simulink library "outp"  (R2021b)
settings: Solver=VariableStepAuto  StartTime=0.0  StopTime=10.0  RelTol=1e-3
undefined symbols (not defined in the file): ENUM_PMMMODE_CHARGE, ENUM_PMMMODE_IDLE, ENUM_PMMMODE_INITIALIZE, ENUM_PMMMODE_POWERDOWN, ENUM_PMMMODE_SLEEP, Left, outp, slcm, TRUE
libraries: FVT_lib x1177, hcu_lib x4, simulink x1
(part 5 of 11)

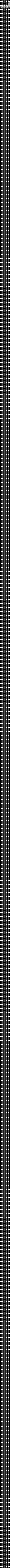
== system outp/OUTP/outpmodule ==
  VACC_HVTHCMSysAvail_enum : Inport
  VACC_LVBattVoltSta_enum : Inport  Port=2
  VACC_VehHVPwrAvail4THCM_W : Inport  Port=3
  VAPM_VehSpeed_kph : Inport  Port=4
  VAPM_VehSpeedTimeOut_flg : Inport  Port=5
  VAPM_FSOffSw_enum : Inport  Port=6
  VAPM_FSOffSwTimeOut_flg : Inport  Port=7
  VAPM_ChrgPlugSta_enum : Inport  Port=8
  VAPM_PASDRMR_cm : Inport  Port=9
  VAPM_PASDRML_cm : Inport  Port=10
  VAPM_PASDRCR_cm : Inport  Port=11
  VAPM_PASDRCL_cm : Inport  Port=12
  VAPM_PASDFMR_cm : Inport  Port=13
  VAPM_PASDFML_cm : Inport  Port=14
  VAPM_PASDFCR_cm : Inport  Port=15
  VAPM_PASDFCL_cm : Inport  Port=16
  VAPM_APSDRLR_cm : Inport  Port=17
  VAPM_APSDRLL_cm : Inport  Port=18
  VAPM_APSDFLR_cm : Inport  Port=19
  VAPM_APSDFLL_cm : Inport  Port=20
  VAPM_PASAFCL_enum : Inport  Port=21
  VAPM_PASARMR_enum : Inport  Port=22
  VAPM_PASARML_enum : Inport  Port=23
  VAPM_PASARCR_enum : Inport  Port=24
  VAPM_PASARCL_enum : Inport  Port=25
  VAPM_PASAFMR_enum : Inport  Port=26
  VAPM_PASAFML_enum : Inport  Port=27
  VAPM_PASAFCR_enum : Inport  Port=28
  VAPM_USSStaRMR_flg : Inport  Port=29
  VAPM_USSStaRML_flg : Inport  Port=30
  VAPM_USSStaRLR_flg : Inport  Port=31
  VAPM_USSStaRLL_flg : Inport  Port=32
  VAPM_USSStaRCR_flg : Inport  Port=33
  VAPM_USSStaRCL_flg : Inport  Port=34
  VAPM_USSStaFMR_flg : Inport  Port=35
  VAPM_USSStaFML_flg : Inport  Port=36
  VAPM_USSStaFLR_flg : Inport  Port=37
  VAPM_USSStaFLL_flg : Inport  Port=38
  VAPM_USSStaFCR_flg : Inport  Port=39
  VAPM_USSStaFCL_flg : Inport  Port=40
  VAPM_Chime_enum : Inport  Port=41
  VAPM_SNSRLayout_enum : Inport  Port=42
  VAPM_StaFSya_flg : Inport  Port=43
  VAPM_ModOperation_enum : Inport  Port=44
  VAPM_BrkPedalPos_pct : Inport  Port=45
  VAPM_BrkPedalPosTimeOut_flg : Inport  Port=46
  VAPM_LFRawWhlSpeed_kph : Inport  Port=47
  VAPM_LFRawWhlSpeedTimeOut_flg : Inport  Port=48
  VAPM_RFRawWhlSpeed_kph : Inport  Port=49
  VAPM_RFRawWhlSpeedTimeOut_flg : Inport  Port=50
  VAPM_LRRawWhlSpeed_kph : Inport  Port=51
  VAPM_LRRawWhlSpeedTimeOut_flg : Inport  Port=52
  VAPM_RRRawWhlSpeed_kph : Inport  Port=53
  VAPM_RRRawWhlSpeedTimeOut_flg : Inport  Port=54
  VAPM_LFRawWhlSpeedV_flg : Inport  Port=55
  VAPM_LFRawWhlSpeedVTimeOut_flg : Inport  Port=56
  VAPM_RFRawWhlSpeedV_flg : Inport  Port=57
  VAPM_RFRawWhlSpeedVTimeOut_flg : Inport  Port=58
  VAPM_LRRawWhlSpeedV_flg : Inport  Port=59
  VAPM_LRRawWhlSpeedVTimeOut_flg : Inport  Port=60
  VAPM_RRRawWhlSpeedV_flg : Inport  Port=61
  VAPM_RRRawWhlSpeedVTimeOut_flg : Inport  Port=62
  VAPM_LFWhlRotDir_enum : Inport  Port=63
  VAPM_LFWhlRotDirTimeOut_flg : Inport  Port=64
  VAPM_RFWhlRotDir_enum : Inport  Port=65
  VAPM_RFWhlRotDirTimeOut_flg : Inport  Port=66
  VAPM_LRWhlRotDir_enum : Inport  Port=67
  VAPM_LRWhlRotDirTimeOut_flg : Inport  Port=68
  VAPM_RRWhlRotDir_enum : Inport  Port=69
  VAPM_RRWhlRotDirTimeOut_flg : Inport  Port=70
  VAPM_LFPulseCountV_flg : Inport  Port=71
  VAPM_LFPulseCountVTimeOut_flg : Inport  Port=72
  VAPM_RFPulseCountV_flg : Inport  Port=73
  VAPM_RFPulseCountVTimeOut_flg : Inport  Port=74
  VAPM_LRPulseCountV_flg : Inport  Port=75
  VAPM_LRPulseCountVTimeOut_flg : Inport  Port=76
  VAPM_RRPulseCountV_flg : Inport  Port=77
  VAPM_RRPulseCountVTimeOut_flg : Inport  Port=78
  VAPM_LFPulseCount_enum : Inport  Port=79
  VAPM_LFPulseCountTimeOut_flg : Inport  Port=80
  VAPM_RFPulseCount_enum : Inport  Port=81
  VAPM_RFPulseCountTimeOut_flg : Inport  Port=82
  VAPM_LRPulseCount_enum : Inport  Port=83
  VAPM_LRPulseCountTimeOut_flg : Inport  Port=84
  VAPM_RRPulseCount_enum : Inport  Port=85
  VAPM_RRPulseCountTimeOut_flg : Inport  Port=86
  VAPM_ShifterHandleCmd_enum : Inport  Port=87
  VAPM_ShifterHandleCmdTimeOut_flg : Inport  Port=88
  VAPM_DriIntend_enum : Inport  Port=89
  VAPM_DriIntendTimeOut_flg : Inport  Port=90
  VAPM_EPSAOIControl_enum : Inport  Port=91
  VAPM_EPSAOIControlTimeOut_flg : Inport  Port=92
  VAPM_SASAngle_Deg : Inport  Port=93
  VAPM_SASAngleTimeOut_flg : Inport  Port=94
  VAPM_SASSpeed_degps : Inport  Port=95
  VAPM_SASSpeedTimeOut_flg : Inport  Port=96
  VAPM_SASSpeedValid_flg : Inport  Port=97
  VAPM_SASSpeedValidTimeOut_flg : Inport  Port=98
  VAPM_SASCAL_flg : Inport  Port=99
  VAPM_SASCALTimeOut_flg : Inport  Port=100
  VAPM_SASV_flg : Inport  Port=101
  VAPM_SASVTimeOut_flg : Inport  Port=102
  VAPM_GRADE_Deg : Inport  Port=103
  VAPM_GRADETimeOut_flg : Inport  Port=104
  VAPM_YawRate_degps : Inport  Port=105
  VAPM_YawRateTimeOut_flg : Inport  Port=106
  VAPM_LatAccel_Gps : Inport  Port=107
  VAPM_LatAccelTimeOut_flg : Inport  Port=108
  VAPM_LongAccel_Gps : Inport  Port=109
  VAPM_LongAccelTimeOut_flg : Inport  Port=110
  VAPM_MCPressure_bar : Inport  Port=111
  VAPM_MCPressureTimeOut_flg : Inport  Port=112
  VAPM_YawRateV_flg : Inport  Port=113
  VAPM_YawRateVTimeOut_flg : Inport  Port=114
  VAPM_LatAccelV_flg : Inport  Port=115
  VAPM_LatAccelVTimeOut_flg : Inport  Port=116
  VAPM_LongAccelV_flg : Inport  Port=117
  VAPM_LongAccelVTimeOut_flg : Inport  Port=118
  VAPM_MCPressureV_bar : Inport  Port=119
  VAPM_MCPressureVTimeOut_flg : Inport  Port=120
  VAPM_BrkSwSta_flg : Inport  Port=121
  VAPM_BrkSwStaTimeOut_flg : Inport  Port=122
  VAPM_BrkSwV_flg : Inport  Port=123
  VAPM_BrkSwVTimeOut_flg : Inport  Port=124
  VAPM_ESCStandstill_flg : Inport  Port=125
  VAPM_ESCStandstillTimeOut_flg : Inport  Port=126
  VAPM_ESCAPSSta_enum : Inport  Port=127
  VAPM_ESCAPSStaTimeOut_flg : Inport  Port=128
  VAPM_EPBExtReleaseAvail_flg : Inport  Port=129
  VAPM_EPBExtReleaseAvailTimeOut_flg : Inport  Port=130
  VAPM_EPBExtApplyAvail_flg : Inport  Port=131
  VAPM_EPBExtApplyAvailTimeOut_flg : Inport  Port=132
  VAPM_EPBErrSta_enum : Inport  Port=133
  VAPM_EPBErrStaTimeOut_flg : Inport  Port=134
  VAPM_EPBSta_enum : Inport  Port=135
  VAPM_EPBStaTimeOut_flg : Inport  Port=136
  VAPM_AVMparkingcancel_enum : Inport  Port=137
  VAPM_AVMparkingcancelTimeOut_flg : Inport  Port=138
  VAPM_AVMparkingexcute_enum : Inport  Port=139
  VAPM_AVMparkingexcuteTimeOut_flg : Inport  Port=140
  VAPM_AVMParkingmode_enum : Inport  Port=141
  VAPM_AVMParkingmodeTimeOut_flg : Inport  Port=142
  VAPM_AVMErrSTA_flg : Inport  Port=143
  VAPM_AVMErrSTATimeOut_flg : Inport  Port=144
  VAPM_IVIStatus_flg : Inport  Port=145
  VAPM_IVIStatusTimeOut_flg : Inport  Port=146
  VAPM_CAASSw_enum : Inport  Port=147
  VAPM_CAASSwTimeOut_flg : Inport  Port=148
  VAPM_IVIScreen_enum : Inport  Port=149
  VAPM_IVIScreenTimeOut_flg : Inport  Port=150
  VAPM_ABSActive_flg : Inport  Port=151
  VAPM_ABSActiveTimeOut_flg : Inport  Port=152
  VAPM_TCSActive_flg : Inport  Port=153
  VAPM_TCSActiveTimeOut_flg : Inport  Port=154
  VAPM_DriverSeatBeltCmd_flg : Inport  Port=155
  VAPM_DriverSeatBeltCmdTimeOut_flg : Inport  Port=156
  VAPM_APSProgressPCT_pct : Inport  Port=157
  VAPM_APSRQDisplay_enum : Inport  Port=158
  VAPM_APSSWVer_enum : Inport  Port=159
  VAPM_APSHWVer_enum : Inport  Port=160
  VAPM_APSExitCondition_enum : Inport  Port=161
  VAPM_APSAngleTarget_Deg : Inport  Port=162
  VAPM_APSVRqEPASCtrl_flg : Inport  Port=163
  VAPM_APSRqEPASCtrl_flg : Inport  Port=164
  VAPM_CAASSta_enum : Inport  Port=165
  VAPM_DKCPDkeyAreaRAPSSta_enum : Inport  Port=166
  VAPM_DKCParkingModeCmd_enum : Inport  Port=167
  VAPM_PUIDLowPower_flg : Inport  Port=168
  VAPM_CAASVMCReqA_flg : Inport  Port=169
  VAPM_APSShiftPosnReq_enum : Inport  Port=170
  VAPM_APSSpeedCMD_kph : Inport  Port=171
  VAPM_APSVMCReqA_flg : Inport  Port=172
  VAPM_RAPSBCMLamp_enum : Inport  Port=173
  VAPM_RAPSBCMLockReq_flg : Inport  Port=174
  VAPM_APSPwrReq_enum : Inport  Port=175
  VAPM_RAPSErrWarnSta_enum : Inport  Port=176
  VAPM_RAPSErrLv1_flg : Inport  Port=177
  VAPM_IVIUserTakeOverAPSSta_flg : Inport  Port=178
  VBCM_AntitheftSta_enum : Inport  Port=179
  VBCM_TailgateRemote_enum : Inport  Port=180
  VBCM_HornCtrl_flg : Inport  Port=181
  VBCM_AllDoorSW_flg : Inport  Port=182
  VBCM_BCMDoorLockSta_flg : Inport  Port=183
  VBCM_AntitheftSeatFlod_flg : Inport  Port=184
  VBCM_HoodSW_flg : Inport  Port=185
  VBCM_TailgateSW_flg : Inport  Port=186
  VBCM_DrDoorSW_flg : Inport  Port=187
  VBCM_PsDoorSW_flg : Inport  Port=188
  VBCM_RLDoorSW_flg : Inport  Port=189
  VBCM_RRDoorSW_flg : Inport  Port=190
  VBCM_LockSetting_flg : Inport  Port=191
  VBCM_FrChargingDoorCtrl_enum : Inport  Port=192
  VBCM_RrChargingDoorCtrl_enum : Inport  Port=193
  VBCM_CrashDetd_flg : Inport  Port=194
  VBCM_CTDCtrl_enum : Inport  Port=195
  VBCM_DoorLockIND_flg : Inport  Port=196
  VBCM_CTDLockSW_flg : Inport  Port=197
  VBCM_Dimmer_pct : Inport  Port=198
  VBCM_DimmerEN_flg : Inport  Port=199
  VBCM_PosLamp_flg : Inport  Port=200
  VBCM_LBeam_flg : Inport  Port=201
  VBCM_HBeam_flg : Inport  Port=202
  VBCM_RrFogLamp_flg : Inport  Port=203
  VBCM_BrakeLamp_flg : Inport  Port=204
  VBCM_ReverseLamp_flg : Inport  Port=205
  VBCM_LDRL_flg : Inport  Port=206
  VBCM_RDRL_flg : Inport  Port=207
  VBCM_LBSD_flg : Inport  Port=208
  VBCM_RBSD_flg : Inport  Port=209
  VBCM_HazardSW_flg : Inport  Port=210
  VBCM_LTurnLP_flg : Inport  Port=211
  VBCM_RTurnLP_flg : Inport  Port=212
  VBCM_BCMBuzzerReq_flg : Inport  Port=213
  VBCM_MirrorCtrl_enum : Inport  Port=214
  VBCM_MirrorDefog_flg : Inport  Port=215
  VBCM_RrDefog_flg : Inport  Port=216
  VBCM_RoomLampH_flg : Inport  Port=217
  VBCM_RoomLampL_flg : Inport  Port=218
  VBCM_TrunkRel_flg : Inport  Port=219
  VBCM_TailgateHDSW_flg : Inport  Port=220
  VBCM_FrWiperL_flg : Inport  Port=221
  VBCM_FrWiperH_flg : Inport  Port=222
  VBCM_RrWiper_flg : Inport  Port=223
  VBCM_WasherCtrl_enum : Inport  Port=224
  VBCM_WiperFixMode_flg : Inport  Port=225
  VBCM_AmbLightBreath1_enum : Inport  Port=226
  VBCM_AmbLightBreath2_enum : Inport  Port=227
  VBCM_AmbLightBreath3_enum : Inport  Port=228
  VBCM_AmbLightBreath4_enum : Inport  Port=229
  VBCM_AmbLightBreath5_enum : Inport  Port=230
  VBCM_AmbLightBreath6_enum : Inport  Port=231
  VBCM_AmbLightBrightness1_enum : Inport  Port=232
  VBCM_AmbLightBrightness2_enum : Inport  Port=233
  VBCM_AmbLightBrightness3_enum : Inport  Port=234
  VBCM_AmbLightBrightness4_enum : Inport  Port=235
  VBCM_AmbLightBrightness5_enum : Inport  Port=236
  VBCM_AmbLightBrightness6_enum : Inport  Port=237
  VBCM_AmbLightColor1_enum : Inport  Port=238
  VBCM_AmbLightColor2_enum : Inport  Port=239
  VBCM_AmbLightColor3_enum : Inport  Port=240
  VBCM_AmbLightColor4_enum : Inport  Port=241
  VBCM_AmbLightColor5_enum : Inport  Port=242
  VBCM_AmbLightColor6_enum : Inport  Port=243
  VBCM_LampPwr_flg : Inport  Port=244
  VBCM_SPTGDet_flg : Inport  Port=245
  VBCM_APSOpenPTG_flg : Inport  Port=246
  VBCM_FollowMe_flg : Inport  Port=247
  VBCM_IVIRST_flg : Inport  Port=248
  VBCM_CountAlarm_enum : Inport  Port=249
  VBCM_MFSWTri_flg : Inport  Port=250
  VBCM_MirrorFlodPos_flg : Inport  Port=251
  VBCM_FuelDoorPos_flg : Inport  Port=252
  VBCM_MFRDNBrightReq_pct : Inport  Port=253
  VBCM_PTGInnerSW2_enum : Inport  Port=254
  VBCM_DrvWdwCtrlCmd_pct : Inport  Port=255
  VBCM_PasWdwCtrlCmd_pct : Inport  Port=256
  VBCM_DrRWdwCtrlCmd_pct : Inport  Port=257
  VBCM_PsRWdwCtrlCmd_pct : Inport  Port=258
  VBCM_APMDoorControlSta_flg : Inport  Port=259
  VBCM_AmbFunEN_flg : Inport  Port=260
  VBCM_AmbWelEN_flg : Inport  Port=261
  VBCM_AmbDimEN_flg : Inport  Port=262
  VBCM_AmbLinkDriSta_flg : Inport  Port=263
  VBCM_AmbPwrWarnEN_flg : Inport  Port=264
  VBCM_AmbODAEN_flg : Inport  Port=265
  VBCM_AmbColorSta_enum : Inport  Port=266
  VBCM_AmbBrightSta_enum : Inport  Port=267
  VBCM_LockAlarm_enum : Inport  Port=268
  VBCM_ATCtrl_enum : Inport  Port=269
  VBCM_fUnlockSingle_flg : Inport  Port=270
  VBCM_UserNow_enum : Inport  Port=271
  VBCM_AmbFunENFlash_enum : Inport  Port=272
  VBCM_AmbWelENFlash_enum : Inport  Port=273
  VBCM_AmbDimENFlash_enum : Inport  Port=274
  VBCM_AmbLinkDriStaFlash_enum : Inport  Port=275
  VBCM_AmbPwrWarnENFlash_enum : Inport  Port=276
  VBCM_AmbODAENFlash_enum : Inport  Port=277
  VBCM_AmbColorSta1_enum : Inport  Port=278
  VBCM_AmbColorSta2_enum : Inport  Port=279
  VBCM_AmbColorSta3_enum : Inport  Port=280
  VBCM_AmbColorSta4_enum : Inport  Port=281
  VBCM_AmbColorSta5_enum : Inport  Port=282
  VBCM_AmbColorSta7_enum : Inport  Port=283
  VBCM_AmbBrightnessSta1_enum : Inport  Port=284
  VBCM_AmbBrightnessSta2_enum : Inport  Port=285
  VBCM_AmbBrightnessSta3_enum : Inport  Port=286
  VBCM_AmbBrightnessSta4_enum : Inport  Port=287
  VBCM_AmbBrightnessSta5_enum : Inport  Port=288
  VBCM_AmbBrightnessSta7_enum : Inport  Port=289
  VBCM_HazardIND_flg : Inport  Port=290
  VBCM_DimSwSta_flg : Inport  Port=291
  VBCM_PassSWSta_flg : Inport  Port=292
  VBCM_FWipSwSta_enum : Inport  Port=293
  VBCM_FWasSwSta_enum : Inport  Port=294
  VBCM_TurnSwSta_enum : Inport  Port=295
  VBCM_TurnSwTSetSta_enum : Inport  Port=296
  VBCM_SPTGENFun_flg : Inport  Port=297
  VBCM_SPTGENFunMem_enum : Inport  Port=298
  VBCM_OutMode_enum : Inport  Port=299
  VBCM_TurnSwTimeSetSta123_enum : Inport  Port=300
  VBCM_TurnSwTimeSetSta457_enum : Inport  Port=301
  VBCM_FDLHandleLampCmd_flg : Inport  Port=302
  VBCM_FDRHandleLampCmd_flg : Inport  Port=303
  VBCM_FDHandleCmd_enum : Inport  Port=304
  VBCM_HBeamADB_enum : Inport  Port=305
  VBCM_WalkInUnLkENMem_enum : Inport  Port=306
  VBCM_WalkOutLkENMem_enum : Inport  Port=307
  VBCM_RmLpModeENMem_enum : Inport  Port=308
  VBCM_LockSettingStaMem_enum : Inport  Port=309
  VBCM_FollowMeENMem_enum : Inport  Port=310
  VBCM_WalkInUnLkENFunSta_flg : Inport  Port=311
  VBCM_WalkOutLkENFunSta_flg : Inport  Port=312
  VBCM_RmLpModeENFunSta_flg : Inport  Port=313
  VBCM_FollowMeENFunSta_flg : Inport  Port=314
  VBCM_HoodRelCmd_flg : Inport  Port=315
  VBCM_WelcomeLight_enum : Inport  Port=316
  VBCM_PTGOpenHeightSta_enum : Inport  Port=317
  VBCM_UserHeightSet_cnt : Inport  Port=318
  VBCM_PTGUserHeight1_cnt : Inport  Port=319
  VBCM_PTGUserHeight2_cnt : Inport  Port=320
  VBCM_PTGUserHeight3_cnt : Inport  Port=321
  VBCM_PTGUserHeight4_cnt : Inport  Port=322
  VBCM_PTGUserHeight5_cnt : Inport  Port=323
  VBCM_PTGUserHeight7_cnt : Inport  Port=324
  VBCM_PTGOpenHeight12_enum : Inport  Port=325
  VBCM_PTGOpenHeight34_enum : Inport  Port=326
  VBCM_PTGOpenHeight57_enum : Inport  Port=327
  VBCM_SenstivityPosnCmd_enum : Inport  Port=328
  VBCM_TimeGapLevelSta_enum : Inport  Port=329
  VBCM_ACCLevelMem12_enum : Inport  Port=330
  VBCM_ACCLevelMem34_enum : Inport  Port=331
  VBCM_ACCLevelMem57_enum : Inport  Port=332
  VBCM_LRightStaCmd_flg : Inport  Port=333
  VBCM_LLeftStaCmd_flg : Inport  Port=334
  VBCM_AutoLockSta_flg : Inport  Port=335
  VBCM_AutoLockMem_enum : Inport  Port=336
  VBCM_AutoUnlockSta_flg : Inport  Port=337
  VBCM_AutoUnlockMem_enum : Inport  Port=338
  VBCM_HMIKey1FuncSta_enum : Inport  Port=339
  VBCM_HMIKey2FuncSta_enum : Inport  Port=340
  VBCM_HMIKey3FuncSta_enum : Inport  Port=341
  VBCM_HMIKey4FuncSta_enum : Inport  Port=342
  VBCM_HMIKey5FuncSta_enum : Inport  Port=343
  VBCM_HMIKey6FuncSta_enum : Inport  Port=344
  VBCM_HMIKey7FuncSta_enum : Inport  Port=345
  VBCM_HMIKey8FuncSta_enum : Inport  Port=346
  VBCM_AutoWipHSpdENSta_flg : Inport  Port=347
  VBCM_DrvWdwReqAP_enum : Inport  Port=348
  VBCM_PasWdwReqAP_enum : Inport  Port=349
  VBCM_DrRWdwReqAP_enum : Inport  Port=350
  VBCM_PsRWdwReqAP_enum : Inport  Port=351
  VBCM_CLWinLockDrSta_flg : Inport  Port=352
  VBCM_CLWinLockDrStaMem_enum : Inport  Port=353
  VBCM_WinLFOpenedSta_pct : Inport  Port=354
  VBCM_WinRFOpenedSta_pct : Inport  Port=355
  VBCM_WinLROpenedSta_pct : Inport  Port=356
  VBCM_WinRROpenedSta_pct : Inport  Port=357
  VDDM_C3BMS6RCDTC_raw32 : Inport  Port=358
  VDDM_C3BMS6CSDTC_raw32 : Inport  Port=359
  VDDM_C3BMS6LCDTC_raw32 : Inport  Port=360
  VDDM_C3BMS1RCDTC_raw32 : Inport  Port=361
  VDDM_C3BMS1CSDTC_raw32 : Inport  Port=362
  VDDM_C3BMS1LCDTC_raw32 : Inport  Port=363
  VDDM_C3CCU1RCDTC_raw32 : Inport  Port=364
  VDDM_C3CCU1CSDTC_raw32 : Inport  Port=365
  VDDM_C3CCU1LCDTC_raw32 : Inport  Port=366
  VDDM_C3CCU2RCDTC_raw32 : Inport  Port=367
  VDDM_C3CCU2CSDTC_raw32 : Inport  Port=368
  VDDM_C3CCU2LCDTC_raw32 : Inport  Port=369
  VDDM_C1ABM1RCDTC_raw32 : Inport  Port=370
  VDDM_C1ABM1CSDTC_raw32 : Inport  Port=371
  VDDM_C1ABM1LCDTC_raw32 : Inport  Port=372
  VDDM_Lv1ErrDTC_raw32 : Inport  Port=373
  VDDM_Lv2ErrDTC_raw32 : Inport  Port=374
  VDDM_Lv3ErrDTC_raw32 : Inport  Port=375
  VDDM_Lv4ErrDTC_raw32 : Inport  Port=376
  VDDM_BrkSWErrDTC_raw32 : Inport  Port=377
  VDDM_BrkSWNoBacDTC_raw32 : Inport  Port=378
  VDDM_KeyAuthDTC_raw32 : Inport  Port=379
  VDDM_ONtoRdyDTC_raw32 : Inport  Port=380
  VDDM_HVB4PreDTC_raw32 : Inport  Port=381
  VDDM_MCU4PreDTC_raw32 : Inport  Port=382
  VDDM_DCDC4PreDTC_raw32 : Inport  Port=383
  VDDM_HVRlyCloDTC_raw32 : Inport  Port=384
  VDDM_BMSRdyDTC_raw32 : Inport  Port=385
  VDDM_DCDCEnaDTC_raw32 : Inport  Port=386
  VDDM_HiLvSaChkDTC_raw32 : Inport  Port=387
  VDDM_MidLvSaChkDTC_raw32 : Inport  Port=388
  VDDM_MCUDisDTC_raw32 : Inport  Port=389
  VDDM_DCDCDisDTC_raw32 : Inport  Port=390
  VDDM_HVRlyOpDTC_raw32 : Inport  Port=391
  VDDM_MCUActDTC_raw32 : Inport  Port=392
  VDDM_OBC4PreDTC_raw32 : Inport  Port=393
  VDDM_IniLVLoDTC_raw32 : Inport  Port=394
  VDDM_LVSupLoDTC_raw32 : Inport  Port=395
  VDDM_LVSupHiDTC_raw32 : Inport  Port=396
  VDDM_DrStSWDTC_raw32 : Inport  Port=397
  VDDM_FLDoorSWDTC_raw32 : Inport  Port=398
  VDDM_RLDoorSWDTC_raw32 : Inport  Port=399
  VDDM_FRDoorSWDTC_raw32 : Inport  Port=400
  VDDM_RRDoorSWDTC_raw32 : Inport  Port=401
  VDDM_HoodSWDTC_raw32 : Inport  Port=402
  VDDM_TailgaSWDTC_raw32 : Inport  Port=403
  VDDM_EDriveSysErrVCUErr_flg : Inport  Port=404
  VDDM_VehMalfunLevel_enum : Inport  Port=405
  VDDM_APS1SigOoRDTC_raw32 : Inport  Port=406
  VDDM_APS2SigOoRDTC_raw32 : Inport  Port=407
  VDDM_APSCorrErrDTC_raw32 : Inport  Port=408
  VDDM_MCUF1NoComDTC_raw32 : Inport  Port=409
  VDDM_MCUR1NoComDTC_raw32 : Inport  Port=410
  VDDM_Shifter1NoComDTC_raw32 : Inport  Port=411
  VDDM_ESC7NoComDTC_raw32 : Inport  Port=412
  VDDM_ESC1NoComDTC_raw32 : Inport  Port=413
  VDDM_ESC5NoComDTC_raw32 : Inport  Port=414
  VDDM_EnterNewOperCyc_flg : Inport  Port=415
  VDDM_DiagHCrashDTC_raw32 : Inport  Port=416
  VDDM_DiagFLTSDTC_raw32 : Inport  Port=417
  VDDM_DiagFRTSDTC_raw32 : Inport  Port=418
  VDDM_DiagRLTSDTC_raw32 : Inport  Port=419
  VDDM_DiagRRTSDTC_raw32 : Inport  Port=420
  VDDM_FCLUSSDTC_raw32 : Inport  Port=421
  VDDM_FMLUSSDTC_raw32 : Inport  Port=422
  VDDM_FMRUSSDTC_raw32 : Inport  Port=423
  VDDM_FCRUSSDTC_raw32 : Inport  Port=424
  VDDM_RCLUSSDTC_raw32 : Inport  Port=425
  VDDM_RMLUSSDTC_raw32 : Inport  Port=426
  VDDM_RMRUSSDTC_raw32 : Inport  Port=427
  VDDM_RCRUSSDTC_raw32 : Inport  Port=428
  VDDM_FLLUSSDTC_raw32 : Inport  Port=429
  VDDM_FLRUSSDTC_raw32 : Inport  Port=430
  VDDM_RLLUSSDTC_raw32 : Inport  Port=431
  VDDM_RLRUSSDTC_raw32 : Inport  Port=432
  VDDM_FCM2NoComDTC_raw32 : Inport  Port=433
  VDDM_FCM2RCErrDTC_raw32 : Inport  Port=434
  VDDM_FCM2CSErrDTC_raw32 : Inport  Port=435
  VDDM_FCM3NoComDTC_raw32 : Inport  Port=436
  VDDM_FCM3RCErrDTC_raw32 : Inport  Port=437
  VDDM_FCM3CSErrDTC_raw32 : Inport  Port=438
  VDDM_FCM4NoComDTC_raw32 : Inport  Port=439
  VDDM_FCM4CSErrDTC_raw32 : Inport  Port=440
  VDDM_FCM5NoComDTC_raw32 : Inport  Port=441
  VDDM_FCM5CSErrDTC_raw32 : Inport  Port=442
  VDDM_ZoneSCPNoComDTC_raw32 : Inport  Port=443
  VDDM_BMSSigErrDetDTC_raw32 : Inport  Port=444
  VDDM_FCMACCSigErrDetDTC_raw32 : Inport  Port=445
  VDDM_FrMCUSigErrDetDTC_raw32 : Inport  Port=446
  VDDM_RrMCUSigErrDetDTC_raw32 : Inport  Port=447
  VDDM_CCUSigErrDetDTC_raw32 : Inport  Port=448
  VDDM_ACCAccelCmdErrDetDTC_raw32 : Inport  Port=449
  VDDM_ACCMalfuncDetDTC_raw32 : Inport  Port=450
  VDDM_CCMalfuncDetDTC_raw32 : Inport  Port=451
  VDDM_MSAMalfuncDetDTC_raw32 : Inport  Port=452
  VDDM_ISAMalfuncDetDTC_raw32 : Inport  Port=453
  VDDM_MCUF1RCErrDTC_raw32 : Inport  Port=454
  VDDM_MCUR1RCErrDTC_raw32 : Inport  Port=455
  VDDM_MCUF1CSErrDTC_raw32 : Inport  Port=456
  VDDM_MCUR1CSErrDTC_raw32 : Inport  Port=457
  VDDM_Shifter1RCErrDTC_raw32 : Inport  Port=458
  VDDM_Shifter1CSErrDTC_raw32 : Inport  Port=459
  VDDM_ESC7RCErrDTC_raw32 : Inport  Port=460
  VDDM_ESC7CSErrDTC_raw32 : Inport  Port=461
  VDDM_ESC1RCErrDTC_raw32 : Inport  Port=462
  VDDM_ESC1CSErrDTC_raw32 : Inport  Port=463
  VDDM_ESC5RCErrDTC_raw32 : Inport  Port=464
  VDDM_ESC5CSErrDTC_raw32 : Inport  Port=465
  VDDM_FrMCUTqErrDTC_raw32 : Inport  Port=466
  VDDM_RrMCUTqErrDTC_raw32 : Inport  Port=467
  VDDM_LFBatwarnDTC_raw32 : Inport  Port=468
  VDDM_RFBatwarnDTC_raw32 : Inport  Port=469
  VDDM_LRBatwarnDTC_raw32 : Inport  Port=470
  VDDM_RRBatwarnDTC_raw32 : Inport  Port=471
  VDDM_LFPressIndiDTC_raw32 : Inport  Port=472
  VDDM_RFPressIndiDTC_raw32 : Inport  Port=473
  VDDM_LRPressIndiDTC_raw32 : Inport  Port=474
  VDDM_RRPressIndiDTC_raw32 : Inport  Port=475
  VDDM_LFWheelTmpHighDTC_raw32 : Inport  Port=476
  VDDM_RFWheelTmpHighDTC_raw32 : Inport  Port=477
  VDDM_LRWheelTmpHighDTC_raw32 : Inport  Port=478
  VDDM_RRWheelTmpHighDTC_raw32 : Inport  Port=479
  VDDM_LFSensorFailDTC_raw32 : Inport  Port=480
  VDDM_RFSensorFailDTC_raw32 : Inport  Port=481
  VDDM_LRSensorFailDTC_raw32 : Inport  Port=482
  VDDM_RRSensorFailDTC_raw32 : Inport  Port=483
  VDDM_C1EPAS2LCDTC_raw32 : Inport  Port=484
  VDDM_5vAPS1PwrErrDTC_raw32 : Inport  Port=485
  VDDM_5vAPS2PwrErrDTC_raw32 : Inport  Port=486
  VDDM_EPBLockTODTC_raw32 : Inport  Port=487
  VDDM_EPBUnlockTODTC_raw32 : Inport  Port=488
  VDDM_LimpHomeAct_flg : Inport  Port=489
  VDDM_DTCDetect_enum : Inport  Port=490
  VDDM_EngagePFail_flg : Inport  Port=491
  VDDM_DisengagePFail_flg : Inport  Port=492
  VDDM_VCURAPSErrLv2_flg : Inport  Port=493
  VDDM_VCURAPSErrLv3_flg : Inport  Port=494
  VDDM_EDriveSysErrShifterErr_flg : Inport  Port=495
  VDDM_LVSysErrPwrOutErr_flg : Inport  Port=496
  VDDM_HVRlyOpFail_flg : Inport  Port=497
  VDDM_MCUActDisFail_flg : Inport  Port=498
  VDDM_VCUBrkSWSta_enum : Inport  Port=499
  VDDM_VCUFLDoorSta_flg : Inport  Port=500
  VDDM_VCUFRDoorSta_flg : Inport  Port=501
  VDDM_VCURLDoorSta_flg : Inport  Port=502
  VDDM_VCURRDoorSta_flg : Inport  Port=503
  VDDM_SysAllowReadySta_flg : Inport  Port=504
  VDDM_VCUHoodSWSta_flg : Inport  Port=505
  VDDM_VCUTailgateSWSta_flg : Inport  Port=506
  VDDM_CAN1BusErrorDTC_raw32 : Inport  Port=507
  VDDM_CAN2BusErrorDTC_raw32 : Inport  Port=508
  VDDM_CAN3BusErrorDTC_raw32 : Inport  Port=509
  VDDM_CAN4BusErrorDTC_raw32 : Inport  Port=510
  VDDM_CAN5BusErrorDTC_raw32 : Inport  Port=511
  VDDM_CAN6BusErrorDTC_raw32 : Inport  Port=512
  VDDM_FrMCU4PreDTC_raw32 : Inport  Port=513
  VDDM_FrMCUDisDTC_raw32 : Inport  Port=514
  VDDM_FrMCUActDTC_raw32 : Inport  Port=515
  VDDM_RegenErrDTC_raw32 : Inport  Port=516
  VDHP_ActAPSPosn_pct : Inport  Port=517
  VDHP_LowIdleAccPedal_flg : Inport  Port=518
  VDHP_EAPS1MIN_pct : Inport  Port=519
  VDHP_EAPS2MIN_pct : Inport  Port=520
  VDHP_ResetPedalZeroPosStart_flg : Inport  Port=521
  VDHP_EAPS1NRM_pct : Inport  Port=522
  VDHP_EAPS2NRM_pct : Inport  Port=523
  VDHP_EAPS1RAW_pct : Inport  Port=524
  VDHP_EAPS2RAW_pct : Inport  Port=525
  VDID_VSS_kph : Inport  Port=526
  VDID_RUNTM_s : Inport  Port=527
  VDID_MILDIST_km : Inport  Port=528
  VDID_CLRDIST_km : Inport  Port=529
  VDID_APPD_pct : Inport  Port=530
  VDID_APPE_pct : Inport  Port=531
  VDID_ODOMETER_km : Inport  Port=532
  VDID_NUMPSATRIPSFLTMEMCLR_cnt : Inport  Port=533
  VDID_PSAR_sec : Inport  Port=534
  VDID_PSAL_sec : Inport  Port=535
  VDID_IPSAR_sec : Inport  Port=536
  VDID_IPSAL_sec : Inport  Port=537
  VDID_CPSAR_sec : Inport  Port=538
  VDID_CPSAL_sec : Inport  Port=539
  VDID_PKER_kphsqr : Inport  Port=540
  VDID_PKEL_kphsqr : Inport  Port=541
  VDID_ResetCDEODTR_km : Inport  Port=542
  VDID_CDEODTR_km : Inport  Port=543
  VDID_CDEODTL_km : Inport  Port=544
  VDID_QTYPSATRIPSR_cnt : Inport  Port=545
  VDID_QTYPSATRIPSL_cnt : Inport  Port=546
  VDID_PROTOCOLID_enum : Inport  Port=547
  VDID_CALID_cnt : Inport  Port=548
  VDID_ECUNAME_cnt : Inport  Port=549
  VDID_PKERNumerator_kphsqr : Inport  Port=550
  VDID_PKELNumerator_kphsqr : Inport  Port=551
  VDID_VinCode_cnt : Inport  Port=552
  VDID_DIDModelVersion_raw : Inport  Port=553
  VDID_DIDModelVersionChksum_raw : Inport  Port=554
  VDKC_DKCTimeSN_cnt : Inport  Port=555
  VDKC_DKCAuthSta_enum : Inport  Port=556
  VDKC_TimeSNDKCFbk_cnt : Inport  Port=557
  VDKC_PCommandToBCM_enum : Inport  Port=558
  VDKC_KeyAreaLockUnlock_enum : Inport  Port=559
  VDKC_KeyMissSta_flg : Inport  Port=560
  VDKC_ShippingMode_flg : Inport  Port=561
  VDKC_KeyNumSta_enum : Inport  Port=562
  VDKC_DkeyShowIVISta_enum : Inport  Port=563
  VDKC_DkeyAreaRAPSSta_enum : Inport  Port=564
  VDKC_KeyAreaPS_enum : Inport  Port=565
  VDKC_KeyAreaSPTGSta_enum : Inport  Port=566
  VDKC_KeyAreaPTG_enum : Inport  Port=567
  VDKC_UWB4Invalid_flg : Inport  Port=568
  VDKC_UWBOnOff_flg : Inport  Port=569
  VDKC_UWB3Invalid_flg : Inport  Port=570
  VDKC_UWB1Invalid_flg : Inport  Port=571
  VDKC_UWB2Invalid_flg : Inport  Port=572
  VDKC_UWB0Invalid_flg : Inport  Port=573
  VDKC_UIDBatVolt_enum : Inport  Port=574
  VDKC_CoordinateX_enum : Inport  Port=575
  VDKC_FDCSPTGDet_flg : Inport  Port=576
  VDKC_FDCSPTGOpen_flg : Inport  Port=577
  VDKC_UIDLowPowerSta_flg : Inport  Port=578
  VDKC_CoordinateY_enum : Inport  Port=579
  VDKC_AllowSleep_flg : Inport  Port=580
  VDKC_KeyTypeSta_enum : Inport  Port=581
  VDKC_CalDistance_enum : Inport  Port=582
  VDKC_UWBDetPTGArea_enum : Inport  Port=583
  VDKC_A0UWBEvent_enum : Inport  Port=584
  VDKC_ParkingModeCmd_enum : Inport  Port=585
  VDKC_KeyModeSta_enum : Inport  Port=586
  VDKC_ReVehData_enum : Inport  Port=587
  VDKC_UWB0Distance_enum : Inport  Port=588
  VDKC_DKeyWelcomeSta_enum : Inport  Port=589
  VDKC_UWB1Distance_enum : Inport  Port=590
  VDKC_UWB2Distance_enum : Inport  Port=591
  VDKC_UWB3Distance_enum : Inport  Port=592
  VDKC_UWB4Distance_enum : Inport  Port=593
  VDKC_BLERSSI_enum : Inport  Port=594
  VDKC_BLEdcEvent_enum : Inport  Port=595
  VDKC_UWB0FPP_enum : Inport  Port=596
  VDKC_UWB1FPP_enum : Inport  Port=597
  VDKC_UWB2FPP_enum : Inport  Port=598
  VDKC_UWB3FPP_enum : Inport  Port=599
  VDKC_UWB4FPP_enum : Inport  Port=600
  VDKC_UWBDetArea_enum : Inport  Port=601
  VDKC_OutputPCMDModule_enum : Inport  Port=602
  VDKC_FDCDKCAllowSleep_flg : Inport  Port=603
  VDKC_JudgeKeepUnlockZone_flg : Inport  Port=604
  VDSC_DISCTurn_flg : Inport  Port=605
  VDSC_DISCTargetSpd_kph : Inport  Port=606
  VDSC_DISCSta_enum : Inport  Port=607
  VDSC_DISCButtSta_flg : Inport  Port=608
  VNMM_AllCANTxReq_flg : Inport  Port=609
  VNMM_NMmTxReq_flg : Inport  Port=610
  VNMM_Awake_enum : Inport  Port=611
  VNMM_CSB_flg : Inport  Port=612
  VNMM_ErrorState_enum : Inport  Port=613
  VNMM_NodeID_enum : Inport  Port=614
  VNMM_PNI_flg : Inport  Port=615
  VNMM_RptMsgReq_flg : Inport  Port=616
  VNMM_WakeUp_enum : Inport  Port=617
  VNMM_ActiveWU_flg : Inport  Port=618
  VNMM_SysNMmSta_enum : Inport  Port=619
  VNMM_NetworkReq_flg : Inport  Port=620
  VPMM_PowerUpState_enum : Inport  Port=621
  VPMM_PowerDownState_enum : Inport  Port=622
  VPMM_PowerUpFault_enum : Inport  Port=623
  VPMM_PowerDownFault_enum : Inport  Port=624
  VPMM_ActiveDischargeReq_flg : Inport  Port=625
  VPMM_DCDCEnaReq_flg : Inport  Port=626
  VPMM_DCDCVoltSetpoint_V : Inport  Port=627
  VPMM_HVBatCnctReq_flg : Inport  Port=628
  VPMM_HVSysReadyToCharge_enum : Inport  Port=629
  VPMM_PowerSta_enum : Inport  Port=630
  VPMM_LVPwrSta_flg : Inport  Port=631
  VPMM_HVPwrSta_flg : Inport  Port=632
  VPMM_SysPowerMode_enum : Inport  Port=633
  VPMM_FrMCUEnaReq_flg : Inport  Port=634
  VPMM_RrMCUEnaReq_flg : Inport  Port=635
  VPMM_DrivetrainSelect_enum : Inport  Port=636
  VPMM_DrSeatSta_enum : Inport  Port=637
  VPMM_PwrStaSelect_enum : Inport  Port=638
  VPMM_PwrStaConstraint_enum : Inport  Port=639
  VPMM_TCountSta_enum : Inport  Port=640
  VPMM_PwrUpReq_enum : Inport  Port=641
  VPMM_PwrDownReq_enum : Inport  Port=642
  VPMM_LowSOCWarn_enum : Inport  Port=643
  VPMM_ReVehThdChkSta_enum : Inport  Port=644
  VPMM_EvccAplusPwrUpReq_flg : Inport  Port=645
  VPMM_PwrStaONTOPopReq_flg : Inport  Port=646
  VPMM_IVIPwrStaONTOPopT_s : Inport  Port=647
  VPMM_LVChrgHoldTtimer_s : Inport  Port=648
  VPMM_LVBattChrgTimeCnt_s : Inport  Port=649
  VPMM_SilentChkAllowSleep_flg : Inport  Port=650
  VPMM_TimerAllowSleep_flg : Inport  Port=651
  VPMM_FDADC12VDetAvg_mV : Inport  Port=652
  VPMM_PMMAllowECUSleep_flg : Inport  Port=653
  VPMM_LVSilentChrgSta_enum : Inport  Port=654
  VPMM_LVSilentChrgReq_flg : Inport  Port=655
  VPMM_LVSilentChrgLv_enum : Inport  Port=656
  VPMM_CtrlFrPwrStbA1P_flg : Inport  Port=657
  VPMM_CtrlFrRC1_flg : Inport  Port=658
  VPMM_CtrlFrBMSCCUCIR_flg : Inport  Port=659
  VPMM_CtrlFrEDUINVERTER_flg : Inport  Port=660
  VPMM_HWResetSta_enum : Inport  Port=661
  VPMM_CtrlDrPwrStbA2_flg : Inport  Port=662
  VPMM_PwrStaTOSta_enum : Inport  Port=663
  VPMM_Sched_ChgTOSta_enum : Inport  Port=664
  VPMM_PwrReq_OTA_enum : Inport  Port=665
  VPMM_OTAPwrReqOFFChkSta_enum : Inport  Port=666
  VPMM_OTAPwrReqStdChkSta_enum : Inport  Port=667
  VPMM_PwrReqRAPSAvail_flg : Inport  Port=668
  VSYS_HWVer1_cnt : Inport  Port=669
  VSYS_HWVer2_cnt : Inport  Port=670
  VSYS_HWVer3_cnt : Inport  Port=671
  VSYS_CarModel1_cnt : Inport  Port=672
  VSYS_CarModel2_cnt : Inport  Port=673
  VSYS_CarModel3_cnt : Inport  Port=674
  VSYS_ECU1_cnt : Inport  Port=675
  VSYS_ECU2_cnt : Inport  Port=676
  VSYS_Major1_cnt : Inport  Port=677
  VSYS_Major2_cnt : Inport  Port=678
  VSYS_Minor1_cnt : Inport  Port=679
  VSYS_Minor2_cnt : Inport  Port=680
  VSYS_Patch1_cnt : Inport  Port=681
  VSYS_Patch2_cnt : Inport  Port=682
  VSYS_Country1_cnt : Inport  Port=683
  VSYS_Country2_cnt : Inport  Port=684
  VSYS_Variation_cnt : Inport  Port=685
  VSYS_Dash1_cnt : Inport  Port=686
  VSYS_Change1_cnt : Inport  Port=687
  VSYS_Change2_cnt : Inport  Port=688
  VSYS_Dash2_cnt : Inport  Port=689
  VSYS_SHA1_cnt : Inport  Port=690
  VSYS_SHA2_cnt : Inport  Port=691
  VSYS_SHA3_cnt : Inport  Port=692
  VSYS_SHA4_cnt : Inport  Port=693
  VSYS_SHA5_cnt : Inport  Port=694
  VSYS_SHA6_cnt : Inport  Port=695
  VSYS_SHA7_cnt : Inport  Port=696
  VSYS_SHA8_cnt : Inport  Port=697
  VSYS_NvWriteReqRisingEdge_flg : Inport  Port=698
  VSYS_FdcSlpReqRisingEdge_flg : Inport  Port=699
  VSYS_FdcSlpTime_sec : Inport  Port=700
  VSYS_PmicBootReason_enum : Inport  Port=701
  VSYS_WisrBootReason_raw32 : Inport  Port=702
  VSYS_AcoreRebootCmdACK_flg : Inport  Port=703
  VSYS_CurrentNmState_enum : Inport  Port=704
  VSYS_ECUGen1_cnt : Inport  Port=705
  VSYS_ECUGen2_cnt : Inport  Port=706
  VSYS_PmicBootPath_raw32 : Inport  Port=707
  VSYS_DrivingMode_cnt : Inport  Port=708
  VSYS_ModelYear_cnt : Inport  Port=709
  VSYS_Var4_cnt : Inport  Port=710
  VSYS_Var5_cnt : Inport  Port=711
  VTHC_FDCompCmd_rpm : Inport  Port=712
  VTHC_FDSOV1Cmd_flg : Inport  Port=713
  VTHC_FDSOV2Cmd_flg : Inport  Port=714
  VTHC_FDSOV3Cmd_flg : Inport  Port=715
  VTHC_FDEXV1Cmd_step : Inport  Port=716
  VTHC_FDEXV2Cmd_step : Inport  Port=717
  VTHC_FDSOTXVCmd_flg : Inport  Port=718
  VTHC_FDFWVCmd_flg : Inport  Port=719
  VTHC_FDTWVCmd_pct : Inport  Port=720
  VTHC_FDFrWPTCHeatPwrCmd_W : Inport  Port=721
  VTHC_CoolgFanActDuty_pct : Inport  Port=722
  VTHC_FDAGSCmd_enum : Inport  Port=723
  VTHC_FDEWP1Cmd_enum : Inport  Port=724
  VTHC_FDEWP2Cmd_enum : Inport  Port=725
  VTHC_FDEWP3Cmd_enum : Inport  Port=726
  VTHC_FDFrLeAPTCHeatPwrCmd_W : Inport  Port=727
  VTHC_FDFrRiAPTCHeatPwrCmd_W : Inport  Port=728
  VTHC_FDRrAPTCHeatPwrCmd_W : Inport  Port=729
  VTHC_FDBlowerCmd_pct : Inport  Port=730
  VTHC_BatteryMode_enum : Inport  Port=731
  VTHC_EDriveMode_enum : Inport  Port=732
  VTHC_CabinMode_enum : Inport  Port=733
  VTHC_CCUACLampSts_flg : Inport  Port=734
  VTHC_CCUAutoLampSts_flg : Inport  Port=735
  VTHC_CCUACMaxLampSts_flg : Inport  Port=736
  VTHC_CCUSyncLampSts_flg : Inport  Port=737
  VTHC_sigAirIntenZon1St_enum : Inport  Port=738
  VTHC_sigWindDirZon1St_enum : Inport  Port=739
  VTHC_sigRecircSt_flg : Inport  Port=740
  VTHC_sigSetTempZon1St_C : Inport  Port=741
  VTHC_sigSetTempZon2St_C : Inport  Port=742
  VTHC_sigClntTHvBattOut_C : Inport  Port=743
  VTHC_sigCbnSolarLeft_W : Inport  Port=744
  VTHC_sigClntTHvBattIn_C : Inport  Port=745
  VTHC_sigCbnSolarRight_W : Inport  Port=746
  VTHC_sigAmbAirT_C : Inport  Port=747
  VTHC_sigCbnAirT_C : Inport  Port=748
  VTHC_ACSubMode_enum : Inport  Port=749
  VTHC_FDRecyAutoCmd_enum : Inport  Port=750
  VTHC_ACModeMem_enum : Inport  Port=751
  VTHC_Face_flg : Inport  Port=752
  VTHC_Foot_flg : Inport  Port=753
  VTHC_Frost_flg : Inport  Port=754
  VTHC_FaceM_flg : Inport  Port=755
  VTHC_FootM_flg : Inport  Port=756
  VTHC_CCUSyncSts_flg : Inport  Port=757
  VTHC_ACForceOFF_flg : Inport  Port=758
  VTHC_RecAutoFlg_flg : Inport  Port=759
  VTHC_AirIntenZone1M_enum : Inport  Port=760
  VTHC_fdefog_flg : Inport  Port=761
  VTHC_sigSetTempZon2StM_C : Inport  Port=762
  VTHC_sigDfrstSt_flg : Inport  Port=763
  VTHC_FDCTHCAirIntZ3Sta_enum : Inport  Port=764
  VTHC_FDCTHCLEVentModeSta_enum : Inport  Port=765
  VTHC_FDCTHCREVentModeSta_enum : Inport  Port=766
  VTHC_FDCTHCLEVentZSta_enum : Inport  Port=767
  VTHC_FDCTHCCLEVentZSta_enum : Inport  Port=768
  VTHC_FDCTHCREVentZSta_enum : Inport  Port=769
  VTHC_FDCTHCCREVentZSta_enum : Inport  Port=770
  VTHC_FDCTHCLEVentYSta_enum : Inport  Port=771
  VTHC_FDCTHCLVentENSta_flg : Inport  Port=772
  VTHC_FDCTHCCLEVentYSta_enum : Inport  Port=773
  VTHC_FDCTHCCLVentENSta_flg : Inport  Port=774
  VTHC_FDCTHCREVentYSta_enum : Inport  Port=775
  VTHC_FDCTHCRVentENSta_flg : Inport  Port=776
  VTHC_FDCTHCCREVentYSta_enum : Inport  Port=777
  VTHC_FDCTHCCRVentENSta_flg : Inport  Port=778
  VTHC_FDCTHCMAPTCForceOFFSta_flg : Inport  Port=779
  VTHC_FDCFGSAirIntSta_enum : Inport  Port=780
  VTHC_FDCFGSChSta_enum : Inport  Port=781
  VTHC_FDCFGSAirIntCmd_enum : Inport  Port=782
  VTHC_FDCFGSFuncSta_enum : Inport  Port=783
  VTHC_FDCFGSChCmd_enum : Inport  Port=784
  VTHC_FDCFGSIONSWSta_flg : Inport  Port=785
  VTHC_FDCFGSIONCmd_flg : Inport  Port=786
  VTHC_FDCTHCMPreWPTCHeatSta_enum : Inport  Port=787
  VTHC_EWPBUflag1_flg : Inport  Port=788
  VTHC_EWPBUflag2_flg : Inport  Port=789
  VTHC_EWPBUflag3_flg : Inport  Port=790
  VTHC_FaceMSet_enum : Inport  Port=791
  VTHC_FootMSet_enum : Inport  Port=792
  VTHC_fdefogSet_enum : Inport  Port=793
  VTHC_CCUSyncStsSet_enum : Inport  Port=794
  VTHC_sigRecircStSet_enum : Inport  Port=795
  VTHC_RecyAutoSet_enum : Inport  Port=796
  VTHC_AirIntenZone1MSet1_enum : Inport  Port=797
  VTHC_AirIntenZone1MSet2_enum : Inport  Port=798
  VTHC_AirIntenZone1MSet3_enum : Inport  Port=799
  VTHC_AirIntenZone1MSet4_enum : Inport  Port=800
  VTHC_AirIntenZone1MSet5_enum : Inport  Port=801
  VTHC_AirIntenZone1MSet7_enum : Inport  Port=802
  VTHC_AirIntenZone3MSet1_enum : Inport  Port=803
  VTHC_AirIntenZone3MSet2_enum : Inport  Port=804
  VTHC_AirIntenZone3MSet3_enum : Inport  Port=805
  VTHC_AirIntenZone3MSet4_enum : Inport  Port=806
  VTHC_AirIntenZone3MSet5_enum : Inport  Port=807
  VTHC_AirIntenZone3MSet7_enum : Inport  Port=808
  VTHC_IONSWStaSet_enum : Inport  Port=809
  VTHC_FDCFGSChStaSet123_enum : Inport  Port=810
  VTHC_FDCFGSChStaSet457_enum : Inport  Port=811
  VTHC_FDCFGSAirIntStaSet123_enum : Inport  Port=812
  VTHC_FDCFGSAirIntStaSet457_enum : Inport  Port=813
  VTHC_LVentENSet_enum : Inport  Port=814
  VTHC_CLVentENSet_enum : Inport  Port=815
  VTHC_RVentENSet_enum : Inport  Port=816
  VTHC_CRVentENSet_enum : Inport  Port=817
  VTHC_LEVentModeStaSet123_enum : Inport  Port=818
  VTHC_LEVentModeStaSet457_enum : Inport  Port=819
  VTHC_REVentModeStaSet123_enum : Inport  Port=820
  VTHC_REVentModeStaSet457_enum : Inport  Port=821
  VTHC_FDCTHCLEVentZStaSet1_enum : Inport  Port=822
  VTHC_FDCTHCLEVentZStaSet2_enum : Inport  Port=823
  VTHC_FDCTHCLEVentZStaSet3_enum : Inport  Port=824
  VTHC_FDCTHCLEVentZStaSet4_enum : Inport  Port=825
  VTHC_FDCTHCLEVentZStaSet5_enum : Inport  Port=826
  VTHC_FDCTHCLEVentZStaSet7_enum : Inport  Port=827
  VTHC_FDCTHCCLEVentZStaSet1_enum : Inport  Port=828
  VTHC_FDCTHCCLEVentZStaSet2_enum : Inport  Port=829
  VTHC_FDCTHCCLEVentZStaSet3_enum : Inport  Port=830
  VTHC_FDCTHCCLEVentZStaSet4_enum : Inport  Port=831
  VTHC_FDCTHCCLEVentZStaSet5_enum : Inport  Port=832
  VTHC_FDCTHCCLEVentZStaSet7_enum : Inport  Port=833
  VTHC_FDCTHCREVentZStaSet1_enum : Inport  Port=834
  VTHC_FDCTHCREVentZStaSet2_enum : Inport  Port=835
  VTHC_FDCTHCREVentZStaSet3_enum : Inport  Port=836
  VTHC_FDCTHCREVentZStaSet4_enum : Inport  Port=837
  VTHC_FDCTHCREVentZStaSet5_enum : Inport  Port=838
  VTHC_FDCTHCREVentZStaSet7_enum : Inport  Port=839
  VTHC_FDCTHCCREVentZStaSet1_enum : Inport  Port=840
  VTHC_FDCTHCCREVentZStaSet2_enum : Inport  Port=841
  VTHC_FDCTHCCREVentZStaSet3_enum : Inport  Port=842
  VTHC_FDCTHCCREVentZStaSet4_enum : Inport  Port=843
  VTHC_FDCTHCCREVentZStaSet5_enum : Inport  Port=844
  VTHC_FDCTHCCREVentZStaSet7_enum : Inport  Port=845
  VTHC_FDCTHCLEVentYStaSet1_enum : Inport  Port=846
  VTHC_FDCTHCLEVentYStaSet2_enum : Inport  Port=847
  VTHC_FDCTHCLEVentYStaSet3_enum : Inport  Port=848
  VTHC_FDCTHCLEVentYStaSet4_enum : Inport  Port=849
  VTHC_FDCTHCLEVentYStaSet5_enum : Inport  Port=850
  VTHC_FDCTHCLEVentYStaSet7_enum : Inport  Port=851
  VTHC_FDCTHCCLEVentYStaSet1_enum : Inport  Port=852
  VTHC_FDCTHCCLEVentYStaSet2_enum : Inport  Port=853
  VTHC_FDCTHCCLEVentYStaSet3_enum : Inport  Port=854
  VTHC_FDCTHCCLEVentYStaSet4_enum : Inport  Port=855
  VTHC_FDCTHCCLEVentYStaSet5_enum : Inport  Port=856
  VTHC_FDCTHCCLEVentYStaSet7_enum : Inport  Port=857
  VTHC_FDCTHCREVentYStaSet1_enum : Inport  Port=858
  VTHC_FDCTHCREVentYStaSet2_enum : Inport  Port=859
  VTHC_FDCTHCREVentYStaSet3_enum : Inport  Port=860
  VTHC_FDCTHCREVentYStaSet4_enum : Inport  Port=861
  VTHC_FDCTHCREVentYStaSet5_enum : Inport  Port=862
  VTHC_FDCTHCREVentYStaSet7_enum : Inport  Port=863
  VTHC_FDCTHCCREVentYStaSet1_enum : Inport  Port=864
  VTHC_FDCTHCCREVentYStaSet2_enum : Inport  Port=865
  VTHC_FDCTHCCREVentYStaSet3_enum : Inport  Port=866
  VTHC_FDCTHCCREVentYStaSet4_enum : Inport  Port=867
  VTHC_FDCTHCCREVentYStaSet5_enum : Inport  Port=868
  VTHC_FDCTHCCREVentYStaSet7_enum : Inport  Port=869
  VTHC_SettempZon1Set1_enum : Inport  Port=870
  VTHC_SettempZon1Set2_enum : Inport  Port=871
  VTHC_SettempZon1Set3_enum : Inport  Port=872
  VTHC_SettempZon1Set4_enum : Inport  Port=873
  VTHC_SettempZon1Set5_enum : Inport  Port=874
  VTHC_SettempZon1Set7_enum : Inport  Port=875
  VTHC_ACModeSet123_enum : Inport  Port=876
  VTHC_ACModeSet457_enum : Inport  Port=877
  VTHC_FACESet_enum : Inport  Port=878
  VTHC_FOOTSet_enum : Inport  Port=879
  VTHC_FrostSet_enum : Inport  Port=880
  VTHC_LVentEN_flg : Inport  Port=881
  VTHC_CLVentEN_flg : Inport  Port=882
  VTHC_RVentEN_flg : Inport  Port=883
  VTHC_CRVentEN_flg : Inport  Port=884
  VTHC_FDCFGSLearnCmd_enum : Inport  Port=885
  VTHC_FDCFGSFuncSta_flg : Inport  Port=886
  VTHC_THSysErrlampReq_flg : Inport  Port=887
  VTPM_LFBatWarn_flg : Inport  Port=888
  VTPM_RFBatWarn_flg : Inport  Port=889
  VTPM_LRBatWarn_flg : Inport  Port=890
  VTPM_RRBatWarn_flg : Inport  Port=891
  VTPM_LFWheelPress_raw8 : Inport  Port=892
  VTPM_RFWheelPress_raw8 : Inport  Port=893
  VTPM_LRWheelPress_raw8 : Inport  Port=894
  VTPM_RRWheelPress_raw8 : Inport  Port=895
  VTPM_LFWheelTemp_C : Inport  Port=896
  VTPM_RFWheelTemp_C : Inport  Port=897
  VTPM_LRWheelTemp_C : Inport  Port=898
  VTPM_RRWheelTemp_C : Inport  Port=899
  VTPM_LFSensorFail_flg : Inport  Port=900
  VTPM_RFSensorFail_flg : Inport  Port=901
  VTPM_LRSensorFail_flg : Inport  Port=902
  VTPM_RRSensorFail_flg : Inport  Port=903
  VTPM_LFWheelDebug_flg : Inport  Port=904
  VTPM_LRWheelDebug_flg : Inport  Port=905
  VTPM_RFWheelDebug_flg : Inport  Port=906
  VTPM_RRWheelDebug_flg : Inport  Port=907
  VTPM_TPMSResButtAllow_flg : Inport  Port=908
  VTPM_TPMSCaliButtAllow_flg : Inport  Port=909
  VTPM_LFPressIndi_enum : Inport  Port=910
  VTPM_RFPressIndi_enum : Inport  Port=911
  VTPM_LRPressIndi_enum : Inport  Port=912
  VTPM_RRPressIndi_enum : Inport  Port=913
  VTPM_TPMSWarnIndi_enum : Inport  Port=914
  VTPM_LFWheelTmpIndi_flg : Inport  Port=915
  VTPM_RFWheelTmpIndi_flg : Inport  Port=916
  VTPM_LRWheelTmpIndi_flg : Inport  Port=917
  VTPM_RRWheelTmpIndi_flg : Inport  Port=918
  VTPM_LFWheelPSW_raw8 : Inport  Port=919
  VTPM_LRWheelPSW_raw8 : Inport  Port=920
  VTPM_RFWheelPSW_raw8 : Inport  Port=921
  VTPM_RRWheelPSW_raw8 : Inport  Port=922
  VTPM_CWheelTips_enum : Inport  Port=923
  VTPM_AutoLTips_enum : Inport  Port=924
  VTPM_LFSensorMode_flg : Inport  Port=925
  VTPM_RFSensorMode_flg : Inport  Port=926
  VTPM_LRSensorMode_flg : Inport  Port=927
  VTPM_RRSensorMode_flg : Inport  Port=928
  VTPM_S1ID_raw32 : Inport  Port=929
  VTPM_S2ID_raw32 : Inport  Port=930
  VTPM_S3ID_raw32 : Inport  Port=931
  VTPM_S4ID_raw32 : Inport  Port=932
  VTPM_S1L_enum : Inport  Port=933
  VTPM_S2L_enum : Inport  Port=934
  VTPM_S3L_enum : Inport  Port=935
  VTPM_S4L_enum : Inport  Port=936
  VTPM_ALFin_flg : Inport  Port=937
  VTPM_LFP20_raw8 : Inport  Port=938
  VTPM_RFP20_raw8 : Inport  Port=939
  VTPM_LRP20_raw8 : Inport  Port=940
  VTPM_RRP20_raw8 : Inport  Port=941
  VTPM_FAT_flg : Inport  Port=942
  VTPM_IDin_raw32 : Inport  Port=943
  VTPM_S1WheelDebugALTU_pct : Inport  Port=944
  VTPM_S2WheelDebugALTU_pct : Inport  Port=945
  VTPM_S3WheelDebugALTU_pct : Inport  Port=946
  VTPM_S4WheelDebugALTU_pct : Inport  Port=947
  VTPM_ID1messageALTU_raw8 : Inport  Port=948
  VTPM_ID2messageALTU_raw8 : Inport  Port=949
  VTPM_ID3messageALTU_raw8 : Inport  Port=950
  VTPM_ID4messageALTU_raw8 : Inport  Port=951
  VTPM_Chkfin_flg : Inport  Port=952
  VTPM_SetIDLoc_flg : Inport  Port=953
  VTPM_TPMSStorge_flg : Inport  Port=954
  VTPM_ChkStorge_flg : Inport  Port=955
  VTPM_TPMSResButt_flg : Inport  Port=956
  VTPM_LFPindi_enum : Inport  Port=957
  VTPM_RFPind_enum : Inport  Port=958
  VTPM_LRPindi_enum : Inport  Port=959
  VTPM_RRPindi_enum : Inport  Port=960
  VTPM_WriteChkLFID_raw : Inport  Port=961
  VTPM_WriteChkRFID_raw : Inport  Port=962
  VTPM_WriteChkLRID_raw : Inport  Port=963
  VTPM_WriteChkRRID_raw : Inport  Port=964
  VTPM_WriteChkfinLFID_raw : Inport  Port=965
  VTPM_WriteChkfinRFID_raw : Inport  Port=966
  VTPM_WriteChkfinLRID_raw : Inport  Port=967
  VTPM_WriteChkfinRRID_raw : Inport  Port=968
  VTPM_Flashchkdatavalid_enum : Inport  Port=969
  VTPM_Flashdatavalid_enum : Inport  Port=970
  VTPM_unlearnSfali_flg : Inport  Port=971
  VTPM_unlearnSfailvalid_enum : Inport  Port=972
  VTPM_Prepresstempvalid_enum : Inport  Port=973
  VTPM_FlashS1ID_raw : Inport  Port=974
  VTPM_FlashS2ID_raw : Inport  Port=975
  VTPM_FlashS3ID_raw : Inport  Port=976
  VTPM_FlashS4ID_raw : Inport  Port=977
  VTPM_FlashIDvalid_enum : Inport  Port=978
  VTPM_WritingCnt_enum : Inport  Port=979
  VTPM_TPMSTLCmd_flg : Inport  Port=980
  VTPM_LProgress_enum : Inport  Port=981
  VTPM_TPMSSensorIDRegStart_flg : Inport  Port=982
  VTPM_ModelVersion_raw : Inport  Port=983
  VTPM_ModelVersionChksum_raw : Inport  Port=984
  VTQD_ParkRequest_flg : Inport  Port=985
  VTQD_TqSourceFr_enum : Inport  Port=986
  VTQD_TqSourceRr_enum : Inport  Port=987
  VTQD_FrEDUAvailBrkRgnTq_Nm : Inport  Port=988
  VTQD_RrEDUAvailBrkRgnTq_Nm : Inport  Port=989
  VTQD_EVDriveMode_enum : Inport  Port=990
  VTQD_ShiftGearPosn_enum : Inport  Port=991
  VTQD_PButtonSta_enum : Inport  Port=992
  VTQD_FrActvDmpDisabReq_flg : Inport  Port=993
  VTQD_RrActvDmpDisabReq_flg : Inport  Port=994
  VTQD_FrRgnDecrSta_flg : Inport  Port=995
  VTQD_RrRgnDecrSta_flg : Inport  Port=996
  VTQD_DriverWhlTqDemFr_Nm : Inport  Port=997
  VTQD_DriverWhlTqDemRr_Nm : Inport  Port=998
  VTQD_FrEDUActTq_Nm : Inport  Port=999
  VTQD_RrEDUActTq_Nm : Inport  Port=1000
  VTQD_FrEDURolRgnTq_Nm : Inport  Port=1001
  VTQD_RrEDURolRgnTq_Nm : Inport  Port=1002
  VTQD_FrEDUSpd_rpm : Inport  Port=1003
  VTQD_RrEDUSpd_rpm : Inport  Port=1004
  VTQD_FrEDUSpdValid_flg : Inport  Port=1005
  VTQD_FrEDUAvailBrkRgnTqV_flg : Inport  Port=1006
  VTQD_RrEDUSpdValid_flg : Inport  Port=1007
  VTQD_RrEDUAvailBrkRgnTqV_flg : Inport  Port=1008
  VTQD_RgnAbnorSta_flg : Inport  Port=1009
  VTQD_PTCSPermSta_flg : Inport  Port=1010
  VTQD_FrRgnPermSta_flg : Inport  Port=1011
  VTQD_RrRgnPermSta_flg : Inport  Port=1012
  VTQD_FrIdcMin_A : Inport  Port=1013
  VTQD_FrIdcMax_A : Inport  Port=1014
  VTQD_FrUdcMin_V : Inport  Port=1015
  VTQD_FrUdcMax_V : Inport  Port=1016
  VTQD_RrIdcMin_A : Inport  Port=1017
  VTQD_RrIdcMax_A : Inport  Port=1018
  VTQD_RrUdcMin_V : Inport  Port=1019
  VTQD_RrUdcMax_V : Inport  Port=1020
  VTQD_ReBrakeLPReq_flg : Inport  Port=1021
  VTQD_BOSEnable_flg : Inport  Port=1022
  VTQD_CreepON_flg : Inport  Port=1023
  VTQD_RDCActive_enum : Inport  Port=1024
  VTQD_EquivAccPedalSWSta_flg : Inport  Port=1025
  VTQD_DriveProtEn_flg : Inport  Port=1026
  VTQD_ActParkRequest_flg : Inport  Port=1027
  VTQD_RegenTqLimitEn_flg : Inport  Port=1028
  VTQD_IVIPwrLockSta_enum : Inport  Port=1029
  VTQD_OPDHoldLamp_flg : Inport  Port=1030
  VTQD_SaveRegenMode_enum : Inport  Port=1031
  VTQD_FDCVCURegenMode_enum : Inport  Port=1032
  VTQD_SpdCtrlMode_enum : Inport  Port=1033
  VTQD_SpdCtrlSta_flg : Inport  Port=1034
  VTQD_SetSpd_kph : Inport  Port=1035
  VTQD_VehActSpd_kph : Inport  Port=1036
  VTQD_RegenLimIndSta_flg : Inport  Port=1037
  VTQD_SetSpdLimWarn_flg : Inport  Port=1038
  VTQD_MaxWhlSlideRate_pct : Inport  Port=1039
  VTQD_TrailerDisOPDSta_flg : Inport  Port=1040
  VTQD_ForceP_flg : Inport  Port=1041
  VTQD_SlideRegenLimTq_Nm : Inport  Port=1042
  VTQD_SimSoundCmd_pct : Inport  Port=1043
  VTQD_SimSouWaveReq_pct : Inport  Port=1044
  VTQR_FrTMTqReq_Nm : Inport  Port=1045
  VTQR_RrTMTqReq_Nm : Inport  Port=1046
  VTQR_FrFirstOrderInpTs_c : Inport  Port=1047
  VTQR_RrFirstOrderInpTs_c : Inport  Port=1048
  VTQR_FrRateLimitInc_Nm : Inport  Port=1049
  VTQR_FrRateLimitDec_Nm : Inport  Port=1050
  VTQR_RrRateLimitInc_Nm : Inport  Port=1051
  VTQR_RrRateLimitDec_Nm : Inport  Port=1052
  VV2L_ReqOBCV2LEna_enum : Inport  Port=1053
  VV2L_ReqV2LIVIPopup_enum : Inport  Port=1054
  VV2L_ReqV2LIVIDisChrg_enum : Inport  Port=1055
  VV2L_ReqOBCExtrV2LEna_enum : Inport  Port=1056
  VV2L_ReqOBCIntrV2LEna_enum : Inport  Port=1057
  VV2L_HVPO120VGrpALDSt_enum : Inport  Port=1058
  VV2L_HVPO120VGrpBLDSt_enum : Inport  Port=1059
  VVMC_FeatSetSpdFinal_raw32 : Inport  Port=1060
  VVMC_VehicleSpeed_mph : Inport  Port=1061
  VVMC_VehicleSpeed_kph : Inport  Port=1062
  VVMC_MeterIndSpeed_raw32 : Inport  Port=1063
  VVMC_VMCAEBCtrlAvail_flg : Inport  Port=1064
  VVMC_VMCACCCtrlAvail_flg : Inport  Port=1065
  VVMC_VMCCCCtrlAvail_flg : Inport  Port=1066
  VVMC_VMCMSACtrlAvail_flg : Inport  Port=1067
  VVMC_FeatArbitrSta_enum : Inport  Port=1068
  VVMC_FeatReqSpd_kph : Inport  Port=1069
  VVMC_JerkPCT_pct : Inport  Port=1070
  VVMC_LimitPCT_pct : Inport  Port=1071
  VVMC_FrontRearSlipRatioCtrl_flg : Inport  Port=1072
  VVMC_RearWhlSlipRatioCtrl_flg : Inport  Port=1073
  VVMC_SingleWhlSlipRatioCtrl_flg : Inport  Port=1074
  VVMC_LatAccCtrl_flg : Inport  Port=1075
  VVMC_SafetyCtrl_flg : Inport  Port=1076
  VVMC_SPD2ACCAct_flg : Inport  Port=1077
  VVMC_AccCalcuPID_mps2 : Inport  Port=1078
  VVMC_ISOAccLimit_mps2 : Inport  Port=1079
  VVMC_ISODecLimit_mps2 : Inport  Port=1080
  VVMC_ISOJerkLimit_mps3 : Inport  Port=1081
  VVMC_ACCRequiredAccel_mps2 : Inport  Port=1082
  VVMC_DISCReqAcc_mps2 : Inport  Port=1083
  VVMC_FeatArbitrFinal_enum : Inport  Port=1084
  VVMC_ActACCRequiredAccel_mps2 : Inport  Port=1085
  VVMC_LateralCtrl_flg : Inport  Port=1086
  VVMC_ADASLKASta_enum : Inport  Port=1087
  VVMC_LKAStrToqReq_Nm : Inport  Port=1088
  VVMC_LKATOIFault_flg : Inport  Port=1089
  VVMC_LKATOIAct_enum : Inport  Port=1090
  VVMC_ADASAEBReq_enum : Inport  Port=1091
  VVMC_ADASFaultSta_flg : Inport  Port=1092
  VVMC_AEBVehHoldReq_flg : Inport  Port=1093
  VVMC_ACCVehHoldReq_flg : Inport  Port=1094
  VVMC_ADASDBSReq_enum : Inport  Port=1095
  VVMC_ADASACCSta_enum : Inport  Port=1096
  VVMC_ACCObjDist_m : Inport  Port=1097
  VVMC_ACCObjRelSpd_mps : Inport  Port=1098
  VVMC_TimeGapLevel_enum : Inport  Port=1099
  VVMC_ACCJerkUpperLimit_mps3 : Inport  Port=1100
  VVMC_ACCComfortBandUpper_mps2 : Inport  Port=1101
  VVMC_ACCJerkLowerLimit_mps3 : Inport  Port=1102
  VVMC_ACCComfortBandLower_mps2 : Inport  Port=1103
  VVMC_ADASVehSpdLim_raw32 : Inport  Port=1104
  VVMC_ADASShftPosnReqA_flg : Inport  Port=1105
  VVMC_ADASShftPosnReq_enum : Inport  Port=1106
  VVMC_ADASForceIdle_flg : Inport  Port=1107
  VVMC_HazardWarningReq_flg : Inport  Port=1108
  VVMC_RightTurnLightReq_flg : Inport  Port=1109
  VVMC_LeftTurnLightReq_flg : Inport  Port=1110
  VVMC_ADASFCWSta_enum : Inport  Port=1111
  VVMC_ADASLDWSta_enum : Inport  Port=1112
  VVMC_ADASFltWrnReq_flg : Inport  Port=1113
  VVMC_ACCObjDstLvl_enum : Inport  Port=1114
  VVMC_ForceLowBeam_enum : Inport  Port=1115
  VVMC_ACCTakeoverReq_flg : Inport  Port=1116
  VVMC_ADASWarningMsg_enum : Inport  Port=1117
  VVMC_ADASCAMSpdLim_enum : Inport  Port=1118
  VVMC_TargetType_enum : Inport  Port=1119
  VVMC_ADASSLIFSpdLim_enum : Inport  Port=1120
  VVMC_LKAHODDisplayWarning_flg : Inport  Port=1121
  VVMC_LKAHODSoundWarning_flg : Inport  Port=1122
  VVMC_ADASLFCSta_enum : Inport  Port=1123
  VVMC_ADASLaneModeL_enum : Inport  Port=1124
  VVMC_ADASLaneModeR_enum : Inport  Port=1125
  VVMC_ADASSLIFSta_enum : Inport  Port=1126
  VVMC_ADASISASta_enum : Inport  Port=1127
  VVMC_ADASLDWMute_flg : Inport  Port=1128
  VVMC_ADASFCWMute_flg : Inport  Port=1129
  VVMC_ADASLFCHandsOffWarning_enum : Inport  Port=1130
  VVMC_LVDADisabled_flg : Inport  Port=1131
  VVMC_LVDAMuteSta_enum : Inport  Port=1132
  VVMC_LVDAFailinfo_flg : Inport  Port=1133
  VVMC_LVDAWarning_flg : Inport  Port=1134
  VVMC_LVDAACCStatusInformation_flg : Inport  Port=1135
  VVMC_ADASLFCWarnSound_enum : Inport  Port=1136
  VVMC_FCMACCmode_enum : Inport  Port=1137
  VVMC_ADASLanetypeR_enum : Inport  Port=1138
  VVMC_ADASLanetypeL_enum : Inport  Port=1139
  VVMC_ADASLanecurveL_raw32 : Inport  Port=1140
  VVMC_ADASLanecurveR_raw32 : Inport  Port=1141
  VVMC_ADASAEBSta_enum : Inport  Port=1142
  VVMC_FCMLDWRequest_enum : Inport  Port=1143
  VVMC_FCMLDWFault_flg : Inport  Port=1144
  VVMC_ACCCtrlAvail_flg : Inport  Port=1145
  VVMC_ACCPedalOvrd_flg : Inport  Port=1146
  VVMC_TimeGapCalcu_s : Inport  Port=1147
  VVMC_CCCtrlSta_enum : Inport  Port=1148
  VVMC_MSACtrlSta_enum : Inport  Port=1149
  VVMC_APSCtrlAvail_flg : Inport  Port=1150
  VVMC_APSActive_flg : Inport  Port=1151
  VVMC_APSStaSys_enum : Inport  Port=1152
  VVMC_APSDecReqA_flg : Inport  Port=1153
  VVMC_APSDecReq_mps2 : Inport  Port=1154
  VVMC_APSReq_enum : Inport  Port=1155
  VVMC_LongAcc_Gps : Inport  Port=1156
  VVMC_CCMSASpdWar_flg : Inport  Port=1157
  VVMC_IMUEnaCmd_flg : Inport  Port=1158
  VVMC_ActStESCYaw_Dps : Inport  Port=1159
  VVMC_CAASCtrlAvail_flg : Inport  Port=1160
  VVMC_CAASActive_flg : Inport  Port=1161
  VVMC_ExtraMSACtrlSta_enum : Inport  Port=1162
  VVMC_CalibratedAccX_G : Inport  Port=1163
  VVMC_CalibratedAccY_G : Inport  Port=1164
  VVMC_CalibratedAccZ_G : Inport  Port=1165
  VVMC_CalibratedGyroX_Dps : Inport  Port=1166
  VVMC_CalibratedGyroY_Dps : Inport  Port=1167
  VVMC_CalibratedGyroZ_Dps : Inport  Port=1168
  VVMC_FDCVMCAPSVRqEPSCtrl_flg : Inport  Port=1169
  VVMC_FDCVMCAPSAngleTarget_deg : Inport  Port=1170
  VVMC_FDCVMCAPSRqEPSCtrl_flg : Inport  Port=1171
  VVMC_FDCVMCAngCtrlTqWtGn_pct : Inport  Port=1172
  VVMC_FDCVMCDrInpTqBstAct_flg : Inport  Port=1173
  VVMC_FDCVMCMaxAngCtrlOutTqLim_Nm : Inport  Port=1174
  VVMC_FDCVMCDrInpTqBstGn_pct : Inport  Port=1175
  VVMC_VehPitchAngleSta_enum : Inport  Port=1176
  VVMC_DMSModeCmd_enum : Inport  Port=1177
  UnitConverter{1..2,6,8..16,21..28,41..42,44,63,65,67,69,79,81,83,85,87,89,91,127,133,135,137,139,141,147,149,158..161,165..167,170,173,175..176,179..180,192..193,195,214,224,226..243,249,253..258,266..269,271..289,293..296,298..301,304..310,316..317,325..332,336,338..346,348..351,353..357,405,490,499,547..549,552..554,556,558..559,562..568,570..573,581..587,589,594..595,601..602,607,611,613..614,617,619,621..624,629..630,633,636..644,654,656,661,663..667,669..697,701,704..706,708..711,723..726,731..733,738..739,749..751,760,764..771,773,775,777,780..784,787,791..880,885,892..895,910..914,919..924,933..936,938..941,948..951,957..960,969..970,972..973,978..979,981,983..984,986..987,990..992,1024,1029,1031..1033,1053..1059,1068,1084,1087,1090..1091,1095..1096,1099,1106,1111..1112,1114..1115,1117..1120,1123..1127,1130,1132,1136..1139,1142..1143,1148..1149,1152,1155,1162,1176..1177} (469 alike) : DataTypeConversion  OutDataTypeStr=uint8
  UnitConverter{5,7,29..40,43,46,48,50,52,54..62,64,66,68,70..78,80,82,84,86,88,90,92,94,96..102,104,106,108,110,112..126,128..132,134,136,138,140,142..146,148,150..156,163..164,168..169,172,174,177..178,181..191,194,196..197,199..213,215..223,225,244..248,250..252,259..265,270,290..292,297,302..303,311..315,333..335,337,347,352,404,415,489,491..498,500..506,518,521,560..561,569,576..578,580,603..605,608..610,612,615..616,618,620,625..626,628,631..632,634..635,645..646,650..651,653,655,657..660,662,668,698..699,703,713..715,718..719,734..737,740,752..759,761,763,772,774,776,778..779,785..786,788..790,881..884,886..891,900..909,915..918,925..928,937,942,952..956,971,980,982,985,993..996,1005..1012,1021..1023,1025..1028,1030,1034,1037..1038,1040..1041,1064..1067,1072..1077,1086,1089,1092..1094,1105,1107..1110,1113,1116,1121..1122,1128..1129,1131,1133..1135,1144..1146,1150..1151,1153,1157..1158,1160..1161,1169,1171,1173} (373 alike) : DataTypeConversion  OutDataTypeStr=boolean
  UnitConverter{3..4,45,47,49,51,53,93,95,103,105,107,109,111,157,162,171,198,517,519..520,522..526,528..532,540..544,550..551,606,627,647..649,652,700,720..722,727..730,741..748,762,896..899,944..947,988..989,997..1004,1013..1020,1035..1036,1039,1042..1052,1060..1063,1069..1071,1078..1083,1085,1088,1097..1098,1100..1104,1140..1141,1147,1154,1156,1159,1163..1168,1170,1172,1174..1175} (139 alike) : DataTypeConversion  OutDataTypeStr=single
  UnitConverter{17..20,318..324,527,533,574,588,590..593,712,716..717} (22 alike) : DataTypeConversion  OutDataTypeStr=uint16
  UnitConverter{358..403,406..414,416..488,507..516,534..539,545..546,555,557,702,707,929..932,943,961..968,974..977} (167 alike) : DataTypeConversion  OutDataTypeStr=uint32
  UnitConverter{575,579,596..600} (7 alike) : DataTypeConversion  OutDataTypeStr=int16
  VACC_HVTHCMSysAvail_enum_Inproc : FVT_lib/outp/OverrideAndLimit  SystemSampleTime=-1  VariantActivationTime=update diagram  Latency=0  AutoFrameSizeCalculation=off
      link override Signal_Limit/_maxval: Value=KOUTP_HVTHCMSysAvail_enum_maxval
      link override Signal_Limit/_minval: Value=KOUTP_HVTHCMSysAvail_enum_minval
      link override Signal_Override/_ovrdflg: Value=KOUTP_HVTHCMSysAvail_enum_ovrdflg
      link override Signal_Override/_ovrdval: Value=KOUTP_HVTHCMSysAvail_enum_ovrdval
  VACC_LVBattVoltSta_enum_Inproc : FVT_lib/outp/OverrideAndLimit  SystemSampleTime=-1  VariantActivationTime=update diagram  Latency=0  AutoFrameSizeCalculation=off
      link override Signal_Limit/_maxval: Value=KOUTP_LVBattVoltSta_enum_maxval
      link override Signal_Limit/_minval: Value=KOUTP_LVBattVoltSta_enum_minval
      link override Signal_Override/_ovrdflg: Value=KOUTP_LVBattVoltSta_enum_ovrdflg
      link override Signal_Override/_ovrdval: Value=KOUTP_LVBattVoltSta_enum_ovrdval
  VACC_VehHVPwrAvail4THCM_W_Inproc : FVT_lib/outp/OverrideAndLimit  SystemSampleTime=-1  VariantActivationTime=update diagram  Latency=0  AutoFrameSizeCalculation=off
      link override Signal_Limit/_maxval: Value=KOUTP_VehHVPwrAvail4THCM_W_maxval
      link override Signal_Limit/_minval: Value=KOUTP_VehHVPwrAvail4THCM_W_minval
      link override Signal_Override/_ovrdflg: Value=KOUTP_VehHVPwrAvail4THCM_W_ovrdflg
      link override Signal_Override/_ovrdval: Value=KOUTP_VehHVPwrAvail4THCM_W_ovrdval
  VAPM_ABSActiveTimeOut_flg_Inproc : FVT_lib/outp/OverrideAndLimit  SystemSampleTime=-1  VariantActivationTime=update diagram  Latency=0  AutoFrameSizeCalculation=off
      link override Signal_Limit/_maxval: Value=KOUTP_ABSActiveTimeOut_flg_maxval
      link override Signal_Limit/_minval: Value=KOUTP_ABSActiveTimeOut_flg_minval
      link override Signal_Override/_ovrdflg: Value=KOUTP_ABSActiveTimeOut_flg_ovrdflg
      link override Signal_Override/_ovrdval: Value=KOUTP_ABSActiveTimeOut_flg_ovrdval
  VAPM_ABSActive_flg_Inproc : FVT_lib/outp/OverrideAndLimit  SystemSampleTime=-1  VariantActivationTime=update diagram  Latency=0  AutoFrameSizeCalculation=off
      link override Signal_Limit/_maxval: Value=KOUTP_ABSActive_flg_maxval
      link override Signal_Limit/_minval: Value=KOUTP_ABSActive_flg_minval
      link override Signal_Override/_ovrdflg: Value=KOUTP_ABSActive_flg_ovrdflg
      link override Signal_Override/_ovrdval: Value=KOUTP_ABSActive_flg_ovrdval
  VAPM_APSAngleTarget_Deg_Inproc : FVT_lib/outp/OverrideAndLimit  SystemSampleTime=-1  VariantActivationTime=update diagram  Latency=0  AutoFrameSizeCalculation=off
      link override Signal_Limit/_maxval: Value=KOUTP_APSAngleTarget_Deg_maxval
      link override Signal_Limit/_minval: Value=KOUTP_APSAngleTarget_Deg_minval
      link override Signal_Override/_ovrdflg: Value=KOUTP_APSAngleTarget_Deg_ovrdflg
      link override Signal_Override/_ovrdval: Value=KOUTP_APSAngleTarget_Deg_ovrdval
  VAPM_APSDFLL_cm_Inproc : FVT_lib/outp/OverrideAndLimit  SystemSampleTime=-1  VariantActivationTime=update diagram  Latency=0  AutoFrameSizeCalculation=off
      link override Signal_Limit/_maxval: Value=KOUTP_APSDFLL_cm_maxval
      link override Signal_Limit/_minval: Value=KOUTP_APSDFLL_cm_minval
      link override Signal_Override/_ovrdflg: Value=KOUTP_APSDFLL_cm_ovrdflg
      link override Signal_Override/_ovrdval: Value=KOUTP_APSDFLL_cm_ovrdval
  VAPM_APSDFLR_cm_Inproc : FVT_lib/outp/OverrideAndLimit  SystemSampleTime=-1  VariantActivationTime=update diagram  Latency=0  AutoFrameSizeCalculation=off
      link override Signal_Limit/_maxval: Value=KOUTP_APSDFLR_cm_maxval
      link override Signal_Limit/_minval: Value=KOUTP_APSDFLR_cm_minval
      link override Signal_Override/_ovrdflg: Value=KOUTP_APSDFLR_cm_ovrdflg
      link override Signal_Override/_ovrdval: Value=KOUTP_APSDFLR_cm_ovrdval
  VAPM_APSDRLL_cm_Inproc : FVT_lib/outp/OverrideAndLimit  SystemSampleTime=-1  VariantActivationTime=update diagram  Latency=0  AutoFrameSizeCalculation=off
      link override Signal_Limit/_maxval: Value=KOUTP_APSDRLL_cm_maxval
      link override Signal_Limit/_minval: Value=KOUTP_APSDRLL_cm_minval
      link override Signal_Override/_ovrdflg: Value=KOUTP_APSDRLL_cm_ovrdflg
      link override Signal_Override/_ovrdval: Value=KOUTP_APSDRLL_cm_ovrdval
  VAPM_APSDRLR_cm_Inproc : FVT_lib/outp/OverrideAndLimit  SystemSampleTime=-1  VariantActivationTime=update diagram  Latency=0  AutoFrameSizeCalculation=off
      link override Signal_Limit/_maxval: Value=KOUTP_APSDRLR_cm_maxval
      link override Signal_Limit/_minval: Value=KOUTP_APSDRLR_cm_minval
      link override Signal_Override/_ovrdflg: Value=KOUTP_APSDRLR_cm_ovrdflg
      link override Signal_Override/_ovrdval: Value=KOUTP_APSDRLR_cm_ovrdval
  VAPM_APSExitCondition_enum_Inproc : FVT_lib/outp/OverrideAndLimit  SystemSampleTime=-1  VariantActivationTime=update diagram  Latency=0  AutoFrameSizeCalculation=off
      link override Signal_Limit/_maxval: Value=KOUTP_APSExitCondition_enum_maxval
      link override Signal_Limit/_minval: Value=KOUTP_APSExitCondition_enum_minval
      link override Signal_Override/_ovrdflg: Value=KOUTP_APSExitCondition_enum_ovrdflg
      link override Signal_Override/_ovrdval: Value=KOUTP_APSExitCondition_enum_ovrdval
  VAPM_APSHWVer_enum_Inproc : FVT_lib/outp/OverrideAndLimit  SystemSampleTime=-1  VariantActivationTime=update diagram  Latency=0  AutoFrameSizeCalculation=off
      link override Signal_Limit/_maxval: Value=KOUTP_APSHWVer_enum_maxval
      link override Signal_Limit/_minval: Value=KOUTP_APSHWVer_enum_minval
      link override Signal_Override/_ovrdflg: Value=KOUTP_APSHWVer_enum_ovrdflg
      link override Signal_Override/_ovrdval: Value=KOUTP_APSHWVer_enum_ovrdval
  VAPM_APSProgressPCT_pct_Inproc : FVT_lib/outp/OverrideAndLimit  SystemSampleTime=-1  VariantActivationTime=update diagram  Latency=0  AutoFrameSizeCalculation=off
      link override Signal_Limit/_maxval: Value=KOUTP_APSProgressPCT_pct_maxval
      link override Signal_Limit/_minval: Value=KOUTP_APSProgressPCT_pct_minval
      link override Signal_Override/_ovrdflg: Value=KOUTP_APSProgressPCT_pct_ovrdflg
      link override Signal_Override/_ovrdval: Value=KOUTP_APSProgressPCT_pct_ovrdval
  VAPM_APSPwrReq_enum_Inproc : FVT_lib/outp/OverrideAndLimit  SystemSampleTime=-1  VariantActivationTime=update diagram  Latency=0  AutoFrameSizeCalculation=off
      link override Signal_Limit/_maxval: Value=KOUTP_APSPwrReq_enum_maxval
      link override Signal_Limit/_minval: Value=KOUTP_APSPwrReq_enum_minval
      link override Signal_Override/_ovrdflg: Value=KOUTP_APSPwrReq_enum_ovrdflg
      link override Signal_Override/_ovrdval: Value=KOUTP_APSPwrReq_enum_ovrdval
  VAPM_APSRQDisplay_enum_Inproc : FVT_lib/outp/OverrideAndLimit  SystemSampleTime=-1  VariantActivationTime=update diagram  Latency=0  AutoFrameSizeCalculation=off
      link override Signal_Limit/_maxval: Value=KOUTP_APSRQDisplay_enum_maxval
      link override Signal_Limit/_minval: Value=KOUTP_APSRQDisplay_enum_minval
      link override Signal_Override/_ovrdflg: Value=KOUTP_APSRQDisplay_enum_ovrdflg
      link override Signal_Override/_ovrdval: Value=KOUTP_APSRQDisplay_enum_ovrdval
  VAPM_APSRqEPASCtrl_flg_Inproc : FVT_lib/outp/OverrideAndLimit  SystemSampleTime=-1  VariantActivationTime=update diagram  Latency=0  AutoFrameSizeCalculation=off
      link override Signal_Limit/_maxval: Value=KOUTP_APSRqEPASCtrl_flg_maxval
      link override Signal_Limit/_minval: Value=KOUTP_APSRqEPASCtrl_flg_minval
      link override Signal_Override/_ovrdflg: Value=KOUTP_APSRqEPASCtrl_flg_ovrdflg
      link override Signal_Override/_ovrdval: Value=KOUTP_APSRqEPASCtrl_flg_ovrdval
  VAPM_APSSWVer_enum_Inproc : FVT_lib/outp/OverrideAndLimit  SystemSampleTime=-1  VariantActivationTime=update diagram  Latency=0  AutoFrameSizeCalculation=off
      link override Signal_Limit/_maxval: Value=KOUTP_APSSWVer_enum_maxval
      link override Signal_Limit/_minval: Value=KOUTP_APSSWVer_enum_minval
      link override Signal_Override/_ovrdflg: Value=KOUTP_APSSWVer_enum_ovrdflg
      link override Signal_Override/_ovrdval: Value=KOUTP_APSSWVer_enum_ovrdval
  VAPM_APSShiftPosnReq_enum_Inproc : FVT_lib/outp/OverrideAndLimit  SystemSampleTime=-1  VariantActivationTime=update diagram  Latency=0  AutoFrameSizeCalculation=off
      link override Signal_Limit/_maxval: Value=KOUTP_APSShiftPosnReq_enum_maxval
      link override Signal_Limit/_minval: Value=KOUTP_APSShiftPosnReq_enum_minval
      link override Signal_Override/_ovrdflg: Value=KOUTP_APSShiftPosnReq_enum_ovrdflg
      link override Signal_Override/_ovrdval: Value=KOUTP_APSShiftPosnReq_enum_ovrdval
  VAPM_APSSpeedCMD_kph_Inproc : FVT_lib/outp/OverrideAndLimit  SystemSampleTime=-1  VariantActivationTime=update diagram  Latency=0  AutoFrameSizeCalculation=off
      link override Signal_Limit/_maxval: Value=KOUTP_APSSpeedCMD_kph_maxval
      link override Signal_Limit/_minval: Value=KOUTP_APSSpeedCMD_kph_minval
      link override Signal_Override/_ovrdflg: Value=KOUTP_APSSpeedCMD_kph_ovrdflg
      link override Signal_Override/_ovrdval: Value=KOUTP_APSSpeedCMD_kph_ovrdval
  VAPM_APSVMCReqA_flg_Inproc : FVT_lib/outp/OverrideAndLimit  SystemSampleTime=-1  VariantActivationTime=update diagram  Latency=0  AutoFrameSizeCalculation=off
      link override Signal_Limit/_maxval: Value=KOUTP_APSVMCReqA_flg_maxval
      link override Signal_Limit/_minval: Value=KOUTP_APSVMCReqA_flg_minval
      link override Signal_Override/_ovrdflg: Value=KOUTP_APSVMCReqA_flg_ovrdflg
      link override Signal_Override/_ovrdval: Value=KOUTP_APSVMCReqA_flg_ovrdval
  VAPM_APSVRqEPASCtrl_flg_Inproc : FVT_lib/outp/OverrideAndLimit  SystemSampleTime=-1  VariantActivationTime=update diagram  Latency=0  AutoFrameSizeCalculation=off
      link override Signal_Limit/_maxval: Value=KOUTP_APSVRqEPASCtrl_flg_maxval
      link override Signal_Limit/_minval: Value=KOUTP_APSVRqEPASCtrl_flg_minval
      link override Signal_Override/_ovrdflg: Value=KOUTP_APSVRqEPASCtrl_flg_ovrdflg
      link override Signal_Override/_ovrdval: Value=KOUTP_APSVRqEPASCtrl_flg_ovrdval
  VAPM_AVMErrSTATimeOut_flg_Inproc : FVT_lib/outp/OverrideAndLimit  SystemSampleTime=-1  VariantActivationTime=update diagram  Latency=0  AutoFrameSizeCalculation=off
      link override Signal_Limit/_maxval: Value=KOUTP_AVMErrSTATimeOut_flg_maxval
      link override Signal_Limit/_minval: Value=KOUTP_AVMErrSTATimeOut_flg_minval
      link override Signal_Override/_ovrdflg: Value=KOUTP_AVMErrSTATimeOut_flg_ovrdflg
      link override Signal_Override/_ovrdval: Value=KOUTP_AVMErrSTATimeOut_flg_ovrdval
  VAPM_AVMErrSTA_flg_Inproc : FVT_lib/outp/OverrideAndLimit  SystemSampleTime=-1  VariantActivationTime=update diagram  Latency=0  AutoFrameSizeCalculation=off
      link override Signal_Limit/_maxval: Value=KOUTP_AVMErrSTA_flg_maxval
      link override Signal_Limit/_minval: Value=KOUTP_AVMErrSTA_flg_minval
      link override Signal_Override/_ovrdflg: Value=KOUTP_AVMErrSTA_flg_ovrdflg
      link override Signal_Override/_ovrdval: Value=KOUTP_AVMErrSTA_flg_ovrdval
  VAPM_AVMParkingmodeTimeOut_flg_Inproc : FVT_lib/outp/OverrideAndLimit  SystemSampleTime=-1  VariantActivationTime=update diagram  Latency=0  AutoFrameSizeCalculation=off
      link override Signal_Limit/_maxval: Value=KOUTP_AVMParkingmodeTimeOut_flg_maxval
      link override Signal_Limit/_minval: Value=KOUTP_AVMParkingmodeTimeOut_flg_minval
      link override Signal_Override/_ovrdflg: Value=KOUTP_AVMParkingmodeTimeOut_flg_ovrdflg
      link override Signal_Override/_ovrdval: Value=KOUTP_AVMParkingmodeTimeOut_flg_ovrdval
  VAPM_AVMParkingmode_enum_Inproc : FVT_lib/outp/OverrideAndLimit  SystemSampleTime=-1  VariantActivationTime=update diagram  Latency=0  AutoFrameSizeCalculation=off
      link override Signal_Limit/_maxval: Value=KOUTP_AVMParkingmode_enum_maxval
      link override Signal_Limit/_minval: Value=KOUTP_AVMParkingmode_enum_minval
      link override Signal_Override/_ovrdflg: Value=KOUTP_AVMParkingmode_enum_ovrdflg
      link override Signal_Override/_ovrdval: Value=KOUTP_AVMParkingmode_enum_ovrdval
  VAPM_AVMparkingcancelTimeOut_flg_Inproc : FVT_lib/outp/OverrideAndLimit  SystemSampleTime=-1  VariantActivationTime=update diagram  Latency=0  AutoFrameSizeCalculation=off
      link override Signal_Limit/_maxval: Value=KOUTP_AVMparkingcancelTimeOut_flg_maxval
      link override Signal_Limit/_minval: Value=KOUTP_AVMparkingcancelTimeOut_flg_minval
      link override Signal_Override/_ovrdflg: Value=KOUTP_AVMparkingcancelTimeOut_flg_ovrdflg
      link override Signal_Override/_ovrdval: Value=KOUTP_AVMparkingcancelTimeOut_flg_ovrdval
  VAPM_AVMparkingcancel_enum_Inproc : FVT_lib/outp/OverrideAndLimit  SystemSampleTime=-1  VariantActivationTime=update diagram  Latency=0  AutoFrameSizeCalculation=off
      link override Signal_Limit/_maxval: Value=KOUTP_AVMparkingcancel_enum_maxval
      link override Signal_Limit/_minval: Value=KOUTP_AVMparkingcancel_enum_minval
      link override Signal_Override/_ovrdflg: Value=KOUTP_AVMparkingcancel_enum_ovrdflg
      link override Signal_Override/_ovrdval: Value=KOUTP_AVMparkingcancel_enum_ovrdval
  VAPM_AVMparkingexcuteTimeOut_flg_Inproc : FVT_lib/outp/OverrideAndLimit  SystemSampleTime=-1  VariantActivationTime=update diagram  Latency=0  AutoFrameSizeCalculation=off
      link override Signal_Limit/_maxval: Value=KOUTP_AVMparkingexcuteTimeOut_flg_maxval
      link override Signal_Limit/_minval: Value=KOUTP_AVMparkingexcuteTimeOut_flg_minval
      link override Signal_Override/_ovrdflg: Value=KOUTP_AVMparkingexcuteTimeOut_flg_ovrdflg
      link override Signal_Override/_ovrdval: Value=KOUTP_AVMparkingexcuteTimeOut_flg_ovrdval
  VAPM_AVMparkingexcute_enum_Inproc : FVT_lib/outp/OverrideAndLimit  SystemSampleTime=-1  VariantActivationTime=update diagram  Latency=0  AutoFrameSizeCalculation=off
      link override Signal_Limit/_maxval: Value=KOUTP_AVMparkingexcute_enum_maxval
      link override Signal_Limit/_minval: Value=KOUTP_AVMparkingexcute_enum_minval
      link override Signal_Override/_ovrdflg: Value=KOUTP_AVMparkingexcute_enum_ovrdflg
      link override Signal_Override/_ovrdval: Value=KOUTP_AVMparkingexcute_enum_ovrdval
  VAPM_BrkPedalPosTimeOut_flg_Inproc : FVT_lib/outp/OverrideAndLimit  SystemSampleTime=-1  VariantActivationTime=update diagram  Latency=0  AutoFrameSizeCalculation=off
      link override Signal_Limit/_maxval: Value=KOUTP_BrkPedalPosTimeOut_flg_maxval
      link override Signal_Limit/_minval: Value=KOUTP_BrkPedalPosTimeOut_flg_minval
      link override Signal_Override/_ovrdflg: Value=KOUTP_BrkPedalPosTimeOut_flg_ovrdflg
      link override Signal_Override/_ovrdval: Value=KOUTP_BrkPedalPosTimeOut_flg_ovrdval
  VAPM_BrkPedalPos_pct_Inproc : FVT_lib/outp/OverrideAndLimit  SystemSampleTime=-1  VariantActivationTime=update diagram  Latency=0  AutoFrameSizeCalculation=off
      link override Signal_Limit/_maxval: Value=KOUTP_BrkPedalPos_pct_maxval
      link override Signal_Limit/_minval: Value=KOUTP_BrkPedalPos_pct_minval
      link override Signal_Override/_ovrdflg: Value=KOUTP_BrkPedalPos_pct_ovrdflg
      link override Signal_Override/_ovrdval: Value=KOUTP_BrkPedalPos_pct_ovrdval
  VAPM_BrkSwStaTimeOut_flg_Inproc : FVT_lib/outp/OverrideAndLimit  SystemSampleTime=-1  VariantActivationTime=update diagram  Latency=0  AutoFrameSizeCalculation=off
      link override Signal_Limit/_maxval: Value=KOUTP_BrkSwStaTimeOut_flg_maxval
      link override Signal_Limit/_minval: Value=KOUTP_BrkSwStaTimeOut_flg_minval
      link override Signal_Override/_ovrdflg: Value=KOUTP_BrkSwStaTimeOut_flg_ovrdflg
      link override Signal_Override/_ovrdval: Value=KOUTP_BrkSwStaTimeOut_flg_ovrdval
  VAPM_BrkSwSta_flg_Inproc : FVT_lib/outp/OverrideAndLimit  SystemSampleTime=-1  VariantActivationTime=update diagram  Latency=0  AutoFrameSizeCalculation=off
      link override Signal_Limit/_maxval: Value=KOUTP_BrkSwSta_flg_maxval
      link override Signal_Limit/_minval: Value=KOUTP_BrkSwSta_flg_minval
      link override Signal_Override/_ovrdflg: Value=KOUTP_BrkSwSta_flg_ovrdflg
      link override Signal_Override/_ovrdval: Value=KOUTP_BrkSwSta_flg_ovrdval
  VAPM_BrkSwVTimeOut_flg_Inproc : FVT_lib/outp/OverrideAndLimit  SystemSampleTime=-1  VariantActivationTime=update diagram  Latency=0  AutoFrameSizeCalculation=off
      link override Signal_Limit/_maxval: Value=KOUTP_BrkSwVTimeOut_flg_maxval
      link override Signal_Limit/_minval: Value=KOUTP_BrkSwVTimeOut_flg_minval
      link override Signal_Override/_ovrdflg: Value=KOUTP_BrkSwVTimeOut_flg_ovrdflg
      link override Signal_Override/_ovrdval: Value=KOUTP_BrkSwVTimeOut_flg_ovrdval
  VAPM_BrkSwV_flg_Inproc : FVT_lib/outp/OverrideAndLimit  SystemSampleTime=-1  VariantActivationTime=update diagram  Latency=0  AutoFrameSizeCalculation=off
      link override Signal_Limit/_maxval: Value=KOUTP_BrkSwV_flg_maxval
      link override Signal_Limit/_minval: Value=KOUTP_BrkSwV_flg_minval
      link override Signal_Override/_ovrdflg: Value=KOUTP_BrkSwV_flg_ovrdflg
      link override Signal_Override/_ovrdval: Value=KOUTP_BrkSwV_flg_ovrdval
  VAPM_CAASSta_enum_Inproc : FVT_lib/outp/OverrideAndLimit  SystemSampleTime=-1  VariantActivationTime=update diagram  Latency=0  AutoFrameSizeCalculation=off
      link override Signal_Limit/_maxval: Value=KOUTP_CAASSta_enum_maxval
      link override Signal_Limit/_minval: Value=KOUTP_CAASSta_enum_minval
      link override Signal_Override/_ovrdflg: Value=KOUTP_CAASSta_enum_ovrdflg
      link override Signal_Override/_ovrdval: Value=KOUTP_CAASSta_enum_ovrdval
  VAPM_CAASSwTimeOut_flg_Inproc : FVT_lib/outp/OverrideAndLimit  SystemSampleTime=-1  VariantActivationTime=update diagram  Latency=0  AutoFrameSizeCalculation=off
      link override Signal_Limit/_maxval: Value=KOUTP_CAASSwTimeOut_flg_maxval
      link override Signal_Limit/_minval: Value=KOUTP_CAASSwTimeOut_flg_minval
      link override Signal_Override/_ovrdflg: Value=KOUTP_CAASSwTimeOut_flg_ovrdflg
      link override Signal_Override/_ovrdval: Value=KOUTP_CAASSwTimeOut_flg_ovrdval
  VAPM_CAASSw_enum_Inproc : FVT_lib/outp/OverrideAndLimit  SystemSampleTime=-1  VariantActivationTime=update diagram  Latency=0  AutoFrameSizeCalculation=off
      link override Signal_Limit/_maxval: Value=KOUTP_CAASSw_enum_maxval
      link override Signal_Limit/_minval: Value=KOUTP_CAASSw_enum_minval
      link override Signal_Override/_ovrdflg: Value=KOUTP_CAASSw_enum_ovrdflg
      link override Signal_Override/_ovrdval: Value=KOUTP_CAASSw_enum_ovrdval
  VAPM_CAASVMCReqA_flg_Inproc : FVT_lib/outp/OverrideAndLimit  SystemSampleTime=-1  VariantActivationTime=update diagram  Latency=0  AutoFrameSizeCalculation=off
      link override Signal_Limit/_maxval: Value=KOUTP_CAASVMCReqA_flg_maxval
      link override Signal_Limit/_minval: Value=KOUTP_CAASVMCReqA_flg_minval
      link override Signal_Override/_ovrdflg: Value=KOUTP_CAASVMCReqA_flg_ovrdflg
      link override Signal_Override/_ovrdval: Value=KOUTP_CAASVMCReqA_flg_ovrdval
  VAPM_Chime_enum_Inproc : FVT_lib/outp/OverrideAndLimit  SystemSampleTime=-1  VariantActivationTime=update diagram  Latency=0  AutoFrameSizeCalculation=off
      link override Signal_Limit/_maxval: Value=KOUTP_Chime_enum_maxval
      link override Signal_Limit/_minval: Value=KOUTP_Chime_enum_minval
      link override Signal_Override/_ovrdflg: Value=KOUTP_Chime_enum_ovrdflg
      link override Signal_Override/_ovrdval: Value=KOUTP_Chime_enum_ovrdval
  VAPM_ChrgPlugSta_enum_Inproc : FVT_lib/outp/OverrideAndLimit  SystemSampleTime=-1  VariantActivationTime=update diagram  Latency=0  AutoFrameSizeCalculation=off
      link override Signal_Limit/_maxval: Value=KOUTP_ChrgPlugSta_enum_maxval
      link override Signal_Limit/_minval: Value=KOUTP_ChrgPlugSta_enum_minval
      link override Signal_Override/_ovrdflg: Value=KOUTP_ChrgPlugSta_enum_ovrdflg
      link override Signal_Override/_ovrdval: Value=KOUTP_ChrgPlugSta_enum_ovrdval
  VAPM_DKCPDkeyAreaRAPSSta_enum_Inproc : FVT_lib/outp/OverrideAndLimit  SystemSampleTime=-1  VariantActivationTime=update diagram  Latency=0  AutoFrameSizeCalculation=off
      link override Signal_Limit/_maxval: Value=KOUTP_DKCPDkeyAreaRAPSSta_enum_maxval
      link override Signal_Limit/_minval: Value=KOUTP_DKCPDkeyAreaRAPSSta_enum_minval
      link override Signal_Override/_ovrdflg: Value=KOUTP_DKCPDkeyAreaRAPSSta_enum_ovrdflg
      link override Signal_Override/_ovrdval: Value=KOUTP_DKCPDkeyAreaRAPSSta_enum_ovrdval
  VAPM_DKCParkingModeCmd_enum_Inproc : FVT_lib/outp/OverrideAndLimit  SystemSampleTime=-1  VariantActivationTime=update diagram  Latency=0  AutoFrameSizeCalculation=off
      link override Signal_Limit/_maxval: Value=KOUTP_DKCParkingModeCmd_enum_maxval
      link override Signal_Limit/_minval: Value=KOUTP_DKCParkingModeCmd_enum_minval
      link override Signal_Override/_ovrdflg: Value=KOUTP_DKCParkingModeCmd_enum_ovrdflg
      link override Signal_Override/_ovrdval: Value=KOUTP_DKCParkingModeCmd_enum_ovrdval
  VAPM_DriIntendTimeOut_flg_Inproc : FVT_lib/outp/OverrideAndLimit  SystemSampleTime=-1  VariantActivationTime=update diagram  Latency=0  AutoFrameSizeCalculation=off
      link override Signal_Limit/_maxval: Value=KOUTP_DriIntendTimeOut_flg_maxval
      link override Signal_Limit/_minval: Value=KOUTP_DriIntendTimeOut_flg_minval
      link override Signal_Override/_ovrdflg: Value=KOUTP_DriIntendTimeOut_flg_ovrdflg
      link override Signal_Override/_ovrdval: Value=KOUTP_DriIntendTimeOut_flg_ovrdval
  VAPM_DriIntend_enum_Inproc : FVT_lib/outp/OverrideAndLimit  SystemSampleTime=-1  VariantActivationTime=update diagram  Latency=0  AutoFrameSizeCalculation=off
      link override Signal_Limit/_maxval: Value=KOUTP_DriIntend_enum_maxval
      link override Signal_Limit/_minval: Value=KOUTP_DriIntend_enum_minval
      link override Signal_Override/_ovrdflg: Value=KOUTP_DriIntend_enum_ovrdflg
      link override Signal_Override/_ovrdval: Value=KOUTP_DriIntend_enum_ovrdval
  VAPM_DriverSeatBeltCmdTimeOut_flg_Inproc : FVT_lib/outp/OverrideAndLimit  SystemSampleTime=-1  VariantActivationTime=update diagram  Latency=0  AutoFrameSizeCalculation=off
      link override Signal_Limit/_maxval: Value=KOUTP_DriverSeatBeltCmdTimeOut_flg_maxval
      link override Signal_Limit/_minval: Value=KOUTP_DriverSeatBeltCmdTimeOut_flg_minval
      link override Signal_Override/_ovrdflg: Value=KOUTP_DriverSeatBeltCmdTimeOut_flg_ovrdflg
      link override Signal_Override/_ovrdval: Value=KOUTP_DriverSeatBeltCmdTimeOut_flg_ovrdval
  VAPM_DriverSeatBeltCmd_flg_Inproc : FVT_lib/outp/OverrideAndLimit  SystemSampleTime=-1  VariantActivationTime=update diagram  Latency=0  AutoFrameSizeCalculation=off
      link override Signal_Limit/_maxval: Value=KOUTP_DriverSeatBeltCmd_flg_maxval
      link override Signal_Limit/_minval: Value=KOUTP_DriverSeatBeltCmd_flg_minval
      link override Signal_Override/_ovrdflg: Value=KOUTP_DriverSeatBeltCmd_flg_ovrdflg
      link override Signal_Override/_ovrdval: Value=KOUTP_DriverSeatBeltCmd_flg_ovrdval
  VAPM_EPBErrStaTimeOut_flg_Inproc : FVT_lib/outp/OverrideAndLimit  SystemSampleTime=-1  VariantActivationTime=update diagram  Latency=0  AutoFrameSizeCalculation=off
      link override Signal_Limit/_maxval: Value=KOUTP_EPBErrStaTimeOut_flg_maxval
      link override Signal_Limit/_minval: Value=KOUTP_EPBErrStaTimeOut_flg_minval
      link override Signal_Override/_ovrdflg: Value=KOUTP_EPBErrStaTimeOut_flg_ovrdflg
      link override Signal_Override/_ovrdval: Value=KOUTP_EPBErrStaTimeOut_flg_ovrdval
  VAPM_EPBErrSta_enum_Inproc : FVT_lib/outp/OverrideAndLimit  SystemSampleTime=-1  VariantActivationTime=update diagram  Latency=0  AutoFrameSizeCalculation=off
      link override Signal_Limit/_maxval: Value=KOUTP_EPBErrSta_enum_maxval
      link override Signal_Limit/_minval: Value=KOUTP_EPBErrSta_enum_minval
      link override Signal_Override/_ovrdflg: Value=KOUTP_EPBErrSta_enum_ovrdflg
      link override Signal_Override/_ovrdval: Value=KOUTP_EPBErrSta_enum_ovrdval
  VAPM_EPBExtApplyAvailTimeOut_flg_Inproc : FVT_lib/outp/OverrideAndLimit  SystemSampleTime=-1  VariantActivationTime=update diagram  Latency=0  AutoFrameSizeCalculation=off
      link override Signal_Limit/_maxval: Value=KOUTP_EPBExtApplyAvailTimeOut_flg_maxval
      link override Signal_Limit/_minval: Value=KOUTP_EPBExtApplyAvailTimeOut_flg_minval
      link override Signal_Override/_ovrdflg: Value=KOUTP_EPBExtApplyAvailTimeOut_flg_ovrdflg
      link override Signal_Override/_ovrdval: Value=KOUTP_EPBExtApplyAvailTimeOut_flg_ovrdval
  VAPM_EPBExtApplyAvail_flg_Inproc : FVT_lib/outp/OverrideAndLimit  SystemSampleTime=-1  VariantActivationTime=update diagram  Latency=0  AutoFrameSizeCalculation=off
      link override Signal_Limit/_maxval: Value=KOUTP_EPBExtApplyAvail_flg_maxval
      link override Signal_Limit/_minval: Value=KOUTP_EPBExtApplyAvail_flg_minval
      link override Signal_Override/_ovrdflg: Value=KOUTP_EPBExtApplyAvail_flg_ovrdflg
      link override Signal_Override/_ovrdval: Value=KOUTP_EPBExtApplyAvail_flg_ovrdval
  VAPM_EPBExtReleaseAvailTimeOut_flg_Inproc : FVT_lib/outp/OverrideAndLimit  SystemSampleTime=-1  VariantActivationTime=update diagram  Latency=0  AutoFrameSizeCalculation=off
      link override Signal_Limit/_maxval: Value=KOUTP_EPBExtReleaseAvailTimeOut_flg_maxval
      link override Signal_Limit/_minval: Value=KOUTP_EPBExtReleaseAvailTimeOut_flg_minval
      link override Signal_Override/_ovrdflg: Value=KOUTP_EPBExtReleaseAvailTimeOut_flg_ovrdflg
      link override Signal_Override/_ovrdval: Value=KOUTP_EPBExtReleaseAvailTimeOut_flg_ovrdval
  VAPM_EPBExtReleaseAvail_flg_Inproc : FVT_lib/outp/OverrideAndLimit  SystemSampleTime=-1  VariantActivationTime=update diagram  Latency=0  AutoFrameSizeCalculation=off
      link override Signal_Limit/_maxval: Value=KOUTP_EPBExtReleaseAvail_flg_maxval
      link override Signal_Limit/_minval: Value=KOUTP_EPBExtReleaseAvail_flg_minval
      link override Signal_Override/_ovrdflg: Value=KOUTP_EPBExtReleaseAvail_flg_ovrdflg
      link override Signal_Override/_ovrdval: Value=KOUTP_EPBExtReleaseAvail_flg_ovrdval
  VAPM_EPBStaTimeOut_flg_Inproc : FVT_lib/outp/OverrideAndLimit  SystemSampleTime=-1  VariantActivationTime=update diagram  Latency=0  AutoFrameSizeCalculation=off
      link override Signal_Limit/_maxval: Value=KOUTP_EPBStaTimeOut_flg_maxval
      link override Signal_Limit/_minval: Value=KOUTP_EPBStaTimeOut_flg_minval
      link override Signal_Override/_ovrdflg: Value=KOUTP_EPBStaTimeOut_flg_ovrdflg
      link override Signal_Override/_ovrdval: Value=KOUTP_EPBStaTimeOut_flg_ovrdval
  VAPM_EPBSta_enum_Inproc : FVT_lib/outp/OverrideAndLimit  SystemSampleTime=-1  VariantActivationTime=update diagram  Latency=0  AutoFrameSizeCalculation=off
      link override Signal_Limit/_maxval: Value=KOUTP_EPBSta_enum_maxval
      link override Signal_Limit/_minval: Value=KOUTP_EPBSta_enum_minval
      link override Signal_Override/_ovrdflg: Value=KOUTP_EPBSta_enum_ovrdflg
      link override Signal_Override/_ovrdval: Value=KOUTP_EPBSta_enum_ovrdval
  VAPM_EPSAOIControlTimeOut_flg_Inproc : FVT_lib/outp/OverrideAndLimit  SystemSampleTime=-1  VariantActivationTime=update diagram  Latency=0  AutoFrameSizeCalculation=off
      link override Signal_Limit/_maxval: Value=KOUTP_EPSAOIControlTimeOut_flg_maxval
      link override Signal_Limit/_minval: Value=KOUTP_EPSAOIControlTimeOut_flg_minval
      link override Signal_Override/_ovrdflg: Value=KOUTP_EPSAOIControlTimeOut_flg_ovrdflg
      link override Signal_Override/_ovrdval: Value=KOUTP_EPSAOIControlTimeOut_flg_ovrdval
  VAPM_EPSAOIControl_enum_Inproc : FVT_lib/outp/OverrideAndLimit  SystemSampleTime=-1  VariantActivationTime=update diagram  Latency=0  AutoFrameSizeCalculation=off
      link override Signal_Limit/_maxval: Value=KOUTP_EPSAOIControl_enum_maxval
      link override Signal_Limit/_minval: Value=KOUTP_EPSAOIControl_enum_minval
      link override Signal_Override/_ovrdflg: Value=KOUTP_EPSAOIControl_enum_ovrdflg
      link override Signal_Override/_ovrdval: Value=KOUTP_EPSAOIControl_enum_ovrdval
  VAPM_ESCAPSStaTimeOut_flg_Inproc : FVT_lib/outp/OverrideAndLimit  SystemSampleTime=-1  VariantActivationTime=update diagram  Latency=0  AutoFrameSizeCalculation=off
      link override Signal_Limit/_maxval: Value=KOUTP_ESCAPSStaTimeOut_flg_maxval
      link override Signal_Limit/_minval: Value=KOUTP_ESCAPSStaTimeOut_flg_minval
      link override Signal_Override/_ovrdflg: Value=KOUTP_ESCAPSStaTimeOut_flg_ovrdflg
      link override Signal_Override/_ovrdval: Value=KOUTP_ESCAPSStaTimeOut_flg_ovrdval
  VAPM_ESCAPSSta_enum_Inproc : FVT_lib/outp/OverrideAndLimit  SystemSampleTime=-1  VariantActivationTime=update diagram  Latency=0  AutoFrameSizeCalculation=off
      link override Signal_Limit/_maxval: Value=KOUTP_ESCAPSSta_enum_maxval
      link override Signal_Limit/_minval: Value=KOUTP_ESCAPSSta_enum_minval
      link override Signal_Override/_ovrdflg: Value=KOUTP_ESCAPSSta_enum_ovrdflg
      link override Signal_Override/_ovrdval: Value=KOUTP_ESCAPSSta_enum_ovrdval
  VAPM_ESCStandstillTimeOut_flg_Inproc : FVT_lib/outp/OverrideAndLimit  SystemSampleTime=-1  VariantActivationTime=update diagram  Latency=0  AutoFrameSizeCalculation=off
      link override Signal_Limit/_maxval: Value=KOUTP_ESCStandstillTimeOut_flg_maxval
      link override Signal_Limit/_minval: Value=KOUTP_ESCStandstillTimeOut_flg_minval
      link override Signal_Override/_ovrdflg: Value=KOUTP_ESCStandstillTimeOut_flg_ovrdflg
      link override Signal_Override/_ovrdval: Value=KOUTP_ESCStandstillTimeOut_flg_ovrdval
  VAPM_ESCStandstill_flg_Inproc : FVT_lib/outp/OverrideAndLimit  SystemSampleTime=-1  VariantActivationTime=update diagram  Latency=0  AutoFrameSizeCalculation=off
      link override Signal_Limit/_maxval: Value=KOUTP_ESCStandstill_flg_maxval
      link override Signal_Limit/_minval: Value=KOUTP_ESCStandstill_flg_minval
      link override Signal_Override/_ovrdflg: Value=KOUTP_ESCStandstill_flg_ovrdflg
      link override Signal_Override/_ovrdval: Value=KOUTP_ESCStandstill_flg_ovrdval
  VAPM_FSOffSwTimeOut_flg_Inproc : FVT_lib/outp/OverrideAndLimit  SystemSampleTime=-1  VariantActivationTime=update diagram  Latency=0  AutoFrameSizeCalculation=off
      link override Signal_Limit/_maxval: Value=KOUTP_FSOffSwTimeOut_flg_maxval
      link override Signal_Limit/_minval: Value=KOUTP_FSOffSwTimeOut_flg_minval
      link override Signal_Override/_ovrdflg: Value=KOUTP_FSOffSwTimeOut_flg_ovrdflg
      link override Signal_Override/_ovrdval: Value=KOUTP_FSOffSwTimeOut_flg_ovrdval
  VAPM_FSOffSw_enum_Inproc : FVT_lib/outp/OverrideAndLimit  SystemSampleTime=-1  VariantActivationTime=update diagram  Latency=0  AutoFrameSizeCalculation=off
      link override Signal_Limit/_maxval: Value=KOUTP_FSOffSw_enum_maxval
      link override Signal_Limit/_minval: Value=KOUTP_FSOffSw_enum_minval
      link override Signal_Override/_ovrdflg: Value=KOUTP_FSOffSw_enum_ovrdflg
      link override Signal_Override/_ovrdval: Value=KOUTP_FSOffSw_enum_ovrdval
  VAPM_GRADETimeOut_flg_Inproc : FVT_lib/outp/OverrideAndLimit  SystemSampleTime=-1  VariantActivationTime=update diagram  Latency=0  AutoFrameSizeCalculation=off
      link override Signal_Limit/_maxval: Value=KOUTP_GRADETimeOut_flg_maxval
      link override Signal_Limit/_minval: Value=KOUTP_GRADETimeOut_flg_minval
      link override Signal_Override/_ovrdflg: Value=KOUTP_GRADETimeOut_flg_ovrdflg
      link override Signal_Override/_ovrdval: Value=KOUTP_GRADETimeOut_flg_ovrdval
  VAPM_GRADE_Deg_Inproc : FVT_lib/outp/OverrideAndLimit  SystemSampleTime=-1  VariantActivationTime=update diagram  Latency=0  AutoFrameSizeCalculation=off
      link override Signal_Limit/_maxval: Value=KOUTP_GRADE_Deg_maxval
      link override Signal_Limit/_minval: Value=KOUTP_GRADE_Deg_minval
      link override Signal_Override/_ovrdflg: Value=KOUTP_GRADE_Deg_ovrdflg
      link override Signal_Override/_ovrdval: Value=KOUTP_GRADE_Deg_ovrdval
  VAPM_IVIScreenTimeOut_flg_Inproc : FVT_lib/outp/OverrideAndLimit  SystemSampleTime=-1  VariantActivationTime=update diagram  Latency=0  AutoFrameSizeCalculation=off
      link override Signal_Limit/_maxval: Value=KOUTP_IVIScreenTimeOut_flg_maxval
      link override Signal_Limit/_minval: Value=KOUTP_IVIScreenTimeOut_flg_minval
      link override Signal_Override/_ovrdflg: Value=KOUTP_IVIScreenTimeOut_flg_ovrdflg
      link override Signal_Override/_ovrdval: Value=KOUTP_IVIScreenTimeOut_flg_ovrdval
  VAPM_IVIScreen_enum_Inproc : FVT_lib/outp/OverrideAndLimit  SystemSampleTime=-1  VariantActivationTime=update diagram  Latency=0  AutoFrameSizeCalculation=off
      link override Signal_Limit/_maxval: Value=KOUTP_IVIScreen_enum_maxval
      link override Signal_Limit/_minval: Value=KOUTP_IVIScreen_enum_minval
      link override Signal_Override/_ovrdflg: Value=KOUTP_IVIScreen_enum_ovrdflg
      link override Signal_Override/_ovrdval: Value=KOUTP_IVIScreen_enum_ovrdval
  VAPM_IVIStatusTimeOut_flg_Inproc : FVT_lib/outp/OverrideAndLimit  SystemSampleTime=-1  VariantActivationTime=update diagram  Latency=0  AutoFrameSizeCalculation=off
      link override Signal_Limit/_maxval: Value=KOUTP_IVIStatusTimeOut_flg_maxval
      link override Signal_Limit/_minval: Value=KOUTP_IVIStatusTimeOut_flg_minval
      link override Signal_Override/_ovrdflg: Value=KOUTP_IVIStatusTimeOut_flg_ovrdflg
      link override Signal_Override/_ovrdval: Value=KOUTP_IVIStatusTimeOut_flg_ovrdval
  VAPM_IVIStatus_flg_Inproc : FVT_lib/outp/OverrideAndLimit  SystemSampleTime=-1  VariantActivationTime=update diagram  Latency=0  AutoFrameSizeCalculation=off
      link override Signal_Limit/_maxval: Value=KOUTP_IVIStatus_flg_maxval
      link override Signal_Limit/_minval: Value=KOUTP_IVIStatus_flg_minval
      link override Signal_Override/_ovrdflg: Value=KOUTP_IVIStatus_flg_ovrdflg
      link override Signal_Override/_ovrdval: Value=KOUTP_IVIStatus_flg_ovrdval
  VAPM_IVIUserTakeOverAPSSta_flg_Inproc : FVT_lib/outp/OverrideAndLimit  SystemSampleTime=-1  VariantActivationTime=update diagram  Latency=0  AutoFrameSizeCalculation=off
      link override Signal_Limit/_maxval: Value=KOUTP_IVIUserTakeOverAPSSta_flg_maxval
      link override Signal_Limit/_minval: Value=KOUTP_IVIUserTakeOverAPSSta_flg_minval
      link override Signal_Override/_ovrdflg: Value=KOUTP_IVIUserTakeOverAPSSta_flg_ovrdflg
      link override Signal_Override/_ovrdval: Value=KOUTP_IVIUserTakeOverAPSSta_flg_ovrdval
  VAPM_LFPulseCountTimeOut_flg_Inproc : FVT_lib/outp/OverrideAndLimit  SystemSampleTime=-1  VariantActivationTime=update diagram  Latency=0  AutoFrameSizeCalculation=off
      link override Signal_Limit/_maxval: Value=KOUTP_LFPulseCountTimeOut_flg_maxval
      link override Signal_Limit/_minval: Value=KOUTP_LFPulseCountTimeOut_flg_minval
      link override Signal_Override/_ovrdflg: Value=KOUTP_LFPulseCountTimeOut_flg_ovrdflg
      link override Signal_Override/_ovrdval: Value=KOUTP_LFPulseCountTimeOut_flg_ovrdval
  VAPM_LFPulseCountVTimeOut_flg_Inproc : FVT_lib/outp/OverrideAndLimit  SystemSampleTime=-1  VariantActivationTime=update diagram  Latency=0  AutoFrameSizeCalculation=off
      link override Signal_Limit/_maxval: Value=KOUTP_LFPulseCountVTimeOut_flg_maxval
      link override Signal_Limit/_minval: Value=KOUTP_LFPulseCountVTimeOut_flg_minval
      link override Signal_Override/_ovrdflg: Value=KOUTP_LFPulseCountVTimeOut_flg_ovrdflg
      link override Signal_Override/_ovrdval: Value=KOUTP_LFPulseCountVTimeOut_flg_ovrdval
  VAPM_LFPulseCountV_flg_Inproc : FVT_lib/outp/OverrideAndLimit  SystemSampleTime=-1  VariantActivationTime=update diagram  Latency=0  AutoFrameSizeCalculation=off
      link override Signal_Limit/_maxval: Value=KOUTP_LFPulseCountV_flg_maxval
      link override Signal_Limit/_minval: Value=KOUTP_LFPulseCountV_flg_minval
      link override Signal_Override/_ovrdflg: Value=KOUTP_LFPulseCountV_flg_ovrdflg
      link override Signal_Override/_ovrdval: Value=KOUTP_LFPulseCountV_flg_ovrdval
  VAPM_LFPulseCount_enum_Inproc : FVT_lib/outp/OverrideAndLimit  SystemSampleTime=-1  VariantActivationTime=update diagram  Latency=0  AutoFrameSizeCalculation=off
      link override Signal_Limit/_maxval: Value=KOUTP_LFPulseCount_enum_maxval
      link override Signal_Limit/_minval: Value=KOUTP_LFPulseCount_enum_minval
      link override Signal_Override/_ovrdflg: Value=KOUTP_LFPulseCount_enum_ovrdflg
      link override Signal_Override/_ovrdval: Value=KOUTP_LFPulseCount_enum_ovrdval
  VAPM_LFRawWhlSpeedTimeOut_flg_Inproc : FVT_lib/outp/OverrideAndLimit  SystemSampleTime=-1  VariantActivationTime=update diagram  Latency=0  AutoFrameSizeCalculation=off
      link override Signal_Limit/_maxval: Value=KOUTP_LFRawWhlSpeedTimeOut_flg_maxval
      link override Signal_Limit/_minval: Value=KOUTP_LFRawWhlSpeedTimeOut_flg_minval
      link override Signal_Override/_ovrdflg: Value=KOUTP_LFRawWhlSpeedTimeOut_flg_ovrdflg
      link override Signal_Override/_ovrdval: Value=KOUTP_LFRawWhlSpeedTimeOut_flg_ovrdval
  VAPM_LFRawWhlSpeedVTimeOut_flg_Inproc : FVT_lib/outp/OverrideAndLimit  SystemSampleTime=-1  VariantActivationTime=update diagram  Latency=0  AutoFrameSizeCalculation=off
      link override Signal_Limit/_maxval: Value=KOUTP_LFRawWhlSpeedVTimeOut_flg_maxval
      link override Signal_Limit/_minval: Value=KOUTP_LFRawWhlSpeedVTimeOut_flg_minval
      link override Signal_Override/_ovrdflg: Value=KOUTP_LFRawWhlSpeedVTimeOut_flg_ovrdflg
      link override Signal_Override/_ovrdval: Value=KOUTP_LFRawWhlSpeedVTimeOut_flg_ovrdval
  VAPM_LFRawWhlSpeedV_flg_Inproc : FVT_lib/outp/OverrideAndLimit  SystemSampleTime=-1  VariantActivationTime=update diagram  Latency=0  AutoFrameSizeCalculation=off
      link override Signal_Limit/_maxval: Value=KOUTP_LFRawWhlSpeedV_flg_maxval
      link override Signal_Limit/_minval: Value=KOUTP_LFRawWhlSpeedV_flg_minval
      link override Signal_Override/_ovrdflg: Value=KOUTP_LFRawWhlSpeedV_flg_ovrdflg
      link override Signal_Override/_ovrdval: Value=KOUTP_LFRawWhlSpeedV_flg_ovrdval
  VAPM_LFRawWhlSpeed_kph_Inproc : FVT_lib/outp/OverrideAndLimit  SystemSampleTime=-1  VariantActivationTime=update diagram  Latency=0  AutoFrameSizeCalculation=off
      link override Signal_Limit/_maxval: Value=KOUTP_LFRawWhlSpeed_kph_maxval
      link override Signal_Limit/_minval: Value=KOUTP_LFRawWhlSpeed_kph_minval
      link override Signal_Override/_ovrdflg: Value=KOUTP_LFRawWhlSpeed_kph_ovrdflg
      link override Signal_Override/_ovrdval: Value=KOUTP_LFRawWhlSpeed_kph_ovrdval
  VAPM_LFWhlRotDirTimeOut_flg_Inproc : FVT_lib/outp/OverrideAndLimit  SystemSampleTime=-1  VariantActivationTime=update diagram  Latency=0  AutoFrameSizeCalculation=off
      link override Signal_Limit/_maxval: Value=KOUTP_LFWhlRotDirTimeOut_flg_maxval
      link override Signal_Limit/_minval: Value=KOUTP_LFWhlRotDirTimeOut_flg_minval
      link override Signal_Override/_ovrdflg: Value=KOUTP_LFWhlRotDirTimeOut_flg_ovrdflg
      link override Signal_Override/_ovrdval: Value=KOUTP_LFWhlRotDirTimeOut_flg_ovrdval
  VAPM_LFWhlRotDir_enum_Inproc : FVT_lib/outp/OverrideAndLimit  SystemSampleTime=-1  VariantActivationTime=update diagram  Latency=0  AutoFrameSizeCalculation=off
      link override Signal_Limit/_maxval: Value=KOUTP_LFWhlRotDir_enum_maxval
      link override Signal_Limit/_minval: Value=KOUTP_LFWhlRotDir_enum_minval
      link override Signal_Override/_ovrdflg: Value=KOUTP_LFWhlRotDir_enum_ovrdflg
      link override Signal_Override/_ovrdval: Value=KOUTP_LFWhlRotDir_enum_ovrdval
  VAPM_LRPulseCountTimeOut_flg_Inproc : FVT_lib/outp/OverrideAndLimit  SystemSampleTime=-1  VariantActivationTime=update diagram  Latency=0  AutoFrameSizeCalculation=off
      link override Signal_Limit/_maxval: Value=KOUTP_LRPulseCountTimeOut_flg_maxval
      link override Signal_Limit/_minval: Value=KOUTP_LRPulseCountTimeOut_flg_minval
      link override Signal_Override/_ovrdflg: Value=KOUTP_LRPulseCountTimeOut_flg_ovrdflg
      link override Signal_Override/_ovrdval: Value=KOUTP_LRPulseCountTimeOut_flg_ovrdval
  VAPM_LRPulseCountVTimeOut_flg_Inproc : FVT_lib/outp/OverrideAndLimit  SystemSampleTime=-1  VariantActivationTime=update diagram  Latency=0  AutoFrameSizeCalculation=off
      link override Signal_Limit/_maxval: Value=KOUTP_LRPulseCountVTimeOut_flg_maxval
      link override Signal_Limit/_minval: Value=KOUTP_LRPulseCountVTimeOut_flg_minval
      link override Signal_Override/_ovrdflg: Value=KOUTP_LRPulseCountVTimeOut_flg_ovrdflg
      link override Signal_Override/_ovrdval: Value=KOUTP_LRPulseCountVTimeOut_flg_ovrdval
  VAPM_LRPulseCountV_flg_Inproc : FVT_lib/outp/OverrideAndLimit  SystemSampleTime=-1  VariantActivationTime=update diagram  Latency=0  AutoFrameSizeCalculation=off
      link override Signal_Limit/_maxval: Value=KOUTP_LRPulseCountV_flg_maxval
      link override Signal_Limit/_minval: Value=KOUTP_LRPulseCountV_flg_minval
      link override Signal_Override/_ovrdflg: Value=KOUTP_LRPulseCountV_flg_ovrdflg
      link override Signal_Override/_ovrdval: Value=KOUTP_LRPulseCountV_flg_ovrdval
  VAPM_LRPulseCount_enum_Inproc : FVT_lib/outp/OverrideAndLimit  SystemSampleTime=-1  VariantActivationTime=update diagram  Latency=0  AutoFrameSizeCalculation=off
      link override Signal_Limit/_maxval: Value=KOUTP_LRPulseCount_enum_maxval
      link override Signal_Limit/_minval: Value=KOUTP_LRPulseCount_enum_minval
      link override Signal_Override/_ovrdflg: Value=KOUTP_LRPulseCount_enum_ovrdflg
      link override Signal_Override/_ovrdval: Value=KOUTP_LRPulseCount_enum_ovrdval
  VAPM_LRRawWhlSpeedTimeOut_flg_Inproc : FVT_lib/outp/OverrideAndLimit  SystemSampleTime=-1  VariantActivationTime=update diagram  Latency=0  AutoFrameSizeCalculation=off
      link override Signal_Limit/_maxval: Value=KOUTP_LRRawWhlSpeedTimeOut_flg_maxval
      link override Signal_Limit/_minval: Value=KOUTP_LRRawWhlSpeedTimeOut_flg_minval
      link override Signal_Override/_ovrdflg: Value=KOUTP_LRRawWhlSpeedTimeOut_flg_ovrdflg
      link override Signal_Override/_ovrdval: Value=KOUTP_LRRawWhlSpeedTimeOut_flg_ovrdval
  VAPM_LRRawWhlSpeedVTimeOut_flg_Inproc : FVT_lib/outp/OverrideAndLimit  SystemSampleTime=-1  VariantActivationTime=update diagram  Latency=0  AutoFrameSizeCalculation=off
      link override Signal_Limit/_maxval: Value=KOUTP_LRRawWhlSpeedVTimeOut_flg_maxval
      link override Signal_Limit/_minval: Value=KOUTP_LRRawWhlSpeedVTimeOut_flg_minval
      link override Signal_Override/_ovrdflg: Value=KOUTP_LRRawWhlSpeedVTimeOut_flg_ovrdflg
      link override Signal_Override/_ovrdval: Value=KOUTP_LRRawWhlSpeedVTimeOut_flg_ovrdval
  VAPM_LRRawWhlSpeedV_flg_Inproc : FVT_lib/outp/OverrideAndLimit  SystemSampleTime=-1  VariantActivationTime=update diagram  Latency=0  AutoFrameSizeCalculation=off
      link override Signal_Limit/_maxval: Value=KOUTP_LRRawWhlSpeedV_flg_maxval
      link override Signal_Limit/_minval: Value=KOUTP_LRRawWhlSpeedV_flg_minval
      link override Signal_Override/_ovrdflg: Value=KOUTP_LRRawWhlSpeedV_flg_ovrdflg
      link override Signal_Override/_ovrdval: Value=KOUTP_LRRawWhlSpeedV_flg_ovrdval
  VAPM_LRRawWhlSpeed_kph_Inproc : FVT_lib/outp/OverrideAndLimit  SystemSampleTime=-1  VariantActivationTime=update diagram  Latency=0  AutoFrameSizeCalculation=off
      link override Signal_Limit/_maxval: Value=KOUTP_LRRawWhlSpeed_kph_maxval
      link override Signal_Limit/_minval: Value=KOUTP_LRRawWhlSpeed_kph_minval
      link override Signal_Override/_ovrdflg: Value=KOUTP_LRRawWhlSpeed_kph_ovrdflg
      link override Signal_Override/_ovrdval: Value=KOUTP_LRRawWhlSpeed_kph_ovrdval
  VAPM_LRWhlRotDirTimeOut_flg_Inproc : FVT_lib/outp/OverrideAndLimit  SystemSampleTime=-1  VariantActivationTime=update diagram  Latency=0  AutoFrameSizeCalculation=off
      link override Signal_Limit/_maxval: Value=KOUTP_LRWhlRotDirTimeOut_flg_maxval
      link override Signal_Limit/_minval: Value=KOUTP_LRWhlRotDirTimeOut_flg_minval
      link override Signal_Override/_ovrdflg: Value=KOUTP_LRWhlRotDirTimeOut_flg_ovrdflg
      link override Signal_Override/_ovrdval: Value=KOUTP_LRWhlRotDirTimeOut_flg_ovrdval
  VAPM_LRWhlRotDir_enum_Inproc : FVT_lib/outp/OverrideAndLimit  SystemSampleTime=-1  VariantActivationTime=update diagram  Latency=0  AutoFrameSizeCalculation=off
      link override Signal_Limit/_maxval: Value=KOUTP_LRWhlRotDir_enum_maxval
      link override Signal_Limit/_minval: Value=KOUTP_LRWhlRotDir_enum_minval
      link override Signal_Override/_ovrdflg: Value=KOUTP_LRWhlRotDir_enum_ovrdflg
      link override Signal_Override/_ovrdval: Value=KOUTP_LRWhlRotDir_enum_ovrdval
  VAPM_LatAccelTimeOut_flg_Inproc : FVT_lib/outp/OverrideAndLimit  SystemSampleTime=-1  VariantActivationTime=update diagram  Latency=0  AutoFrameSizeCalculation=off
      link override Signal_Limit/_maxval: Value=KOUTP_LatAccelTimeOut_flg_maxval
      link override Signal_Limit/_minval: Value=KOUTP_LatAccelTimeOut_flg_minval
      link override Signal_Override/_ovrdflg: Value=KOUTP_LatAccelTimeOut_flg_ovrdflg
      link override Signal_Override/_ovrdval: Value=KOUTP_LatAccelTimeOut_flg_ovrdval
  VAPM_LatAccelVTimeOut_flg_Inproc : FVT_lib/outp/OverrideAndLimit  SystemSampleTime=-1  VariantActivationTime=update diagram  Latency=0  AutoFrameSizeCalculation=off
      link override Signal_Limit/_maxval: Value=KOUTP_LatAccelVTimeOut_flg_maxval
      link override Signal_Limit/_minval: Value=KOUTP_LatAccelVTimeOut_flg_minval
      link override Signal_Override/_ovrdflg: Value=KOUTP_LatAccelVTimeOut_flg_ovrdflg
      link override Signal_Override/_ovrdval: Value=KOUTP_LatAccelVTimeOut_flg_ovrdval
  VAPM_LatAccelV_flg_Inproc : FVT_lib/outp/OverrideAndLimit  SystemSampleTime=-1  VariantActivationTime=update diagram  Latency=0  AutoFrameSizeCalculation=off
      link override Signal_Limit/_maxval: Value=KOUTP_LatAccelV_flg_maxval
      link override Signal_Limit/_minval: Value=KOUTP_LatAccelV_flg_minval
      link override Signal_Override/_ovrdflg: Value=KOUTP_LatAccelV_flg_ovrdflg
      link override Signal_Override/_ovrdval: Value=KOUTP_LatAccelV_flg_ovrdval
  VAPM_LatAccel_Gps_Inproc : FVT_lib/outp/OverrideAndLimit  SystemSampleTime=-1  VariantActivationTime=update diagram  Latency=0  AutoFrameSizeCalculation=off
      link override Signal_Limit/_maxval: Value=KOUTP_LatAccel_Gps_maxval
      link override Signal_Limit/_minval: Value=KOUTP_LatAccel_Gps_minval
      link override Signal_Override/_ovrdflg: Value=KOUTP_LatAccel_Gps_ovrdflg
      link override Signal_Override/_ovrdval: Value=KOUTP_LatAccel_Gps_ovrdval
  VAPM_LongAccelTimeOut_flg_Inproc : FVT_lib/outp/OverrideAndLimit  SystemSampleTime=-1  VariantActivationTime=update diagram  Latency=0  AutoFrameSizeCalculation=off
      link override Signal_Limit/_maxval: Value=KOUTP_LongAccelTimeOut_flg_maxval
      link override Signal_Limit/_minval: Value=KOUTP_LongAccelTimeOut_flg_minval
      link override Signal_Override/_ovrdflg: Value=KOUTP_LongAccelTimeOut_flg_ovrdflg
      link override Signal_Override/_ovrdval: Value=KOUTP_LongAccelTimeOut_flg_ovrdval
  VAPM_LongAccelVTimeOut_flg_Inproc : FVT_lib/outp/OverrideAndLimit  SystemSampleTime=-1  VariantActivationTime=update diagram  Latency=0  AutoFrameSizeCalculation=off
      link override Signal_Limit/_maxval: Value=KOUTP_LongAccelVTimeOut_flg_maxval
      link override Signal_Limit/_minval: Value=KOUTP_LongAccelVTimeOut_flg_minval
      link override Signal_Override/_ovrdflg: Value=KOUTP_LongAccelVTimeOut_flg_ovrdflg
      link override Signal_Override/_ovrdval: Value=KOUTP_LongAccelVTimeOut_flg_ovrdval
  VAPM_LongAccelV_flg_Inproc : FVT_lib/outp/OverrideAndLimit  SystemSampleTime=-1  VariantActivationTime=update diagram  Latency=0  AutoFrameSizeCalculation=off
      link override Signal_Limit/_maxval: Value=KOUTP_LongAccelV_flg_maxval
      link override Signal_Limit/_minval: Value=KOUTP_LongAccelV_flg_minval
      link override Signal_Override/_ovrdflg: Value=KOUTP_LongAccelV_flg_ovrdflg
      link override Signal_Override/_ovrdval: Value=KOUTP_LongAccelV_flg_ovrdval
  VAPM_LongAccel_Gps_Inproc : FVT_lib/outp/OverrideAndLimit  SystemSampleTime=-1  VariantActivationTime=update diagram  Latency=0  AutoFrameSizeCalculation=off
      link override Signal_Limit/_maxval: Value=KOUTP_LongAccel_Gps_maxval
      link override Signal_Limit/_minval: Value=KOUTP_LongAccel_Gps_minval
      link override Signal_Override/_ovrdflg: Value=KOUTP_LongAccel_Gps_ovrdflg
      link override Signal_Override/_ovrdval: Value=KOUTP_LongAccel_Gps_ovrdval
  VAPM_MCPressureTimeOut_flg_Inproc : FVT_lib/outp/OverrideAndLimit  SystemSampleTime=-1  VariantActivationTime=update diagram  Latency=0  AutoFrameSizeCalculation=off
      link override Signal_Limit/_maxval: Value=KOUTP_MCPressureTimeOut_flg_maxval
      link override Signal_Limit/_minval: Value=KOUTP_MCPressureTimeOut_flg_minval
      link override Signal_Override/_ovrdflg: Value=KOUTP_MCPressureTimeOut_flg_ovrdflg
      link override Signal_Override/_ovrdval: Value=KOUTP_MCPressureTimeOut_flg_ovrdval
  VAPM_MCPressureVTimeOut_flg_Inproc : FVT_lib/outp/OverrideAndLimit  SystemSampleTime=-1  VariantActivationTime=update diagram  Latency=0  AutoFrameSizeCalculation=off
      link override Signal_Limit/_maxval: Value=KOUTP_MCPressureVTimeOut_flg_maxval
      link override Signal_Limit/_minval: Value=KOUTP_MCPressureVTimeOut_flg_minval
      link override Signal_Override/_ovrdflg: Value=KOUTP_MCPressureVTimeOut_flg_ovrdflg
      link override Signal_Override/_ovrdval: Value=KOUTP_MCPressureVTimeOut_flg_ovrdval
  VAPM_MCPressureV_bar_Inproc : FVT_lib/outp/OverrideAndLimit  SystemSampleTime=-1  VariantActivationTime=update diagram  Latency=0  AutoFrameSizeCalculation=off
      link override Signal_Limit/_maxval: Value=KOUTP_MCPressureV_bar_maxval
      link override Signal_Limit/_minval: Value=KOUTP_MCPressureV_bar_minval
      link override Signal_Override/_ovrdflg: Value=KOUTP_MCPressureV_bar_ovrdflg
      link override Signal_Override/_ovrdval: Value=KOUTP_MCPressureV_bar_ovrdval
  VAPM_MCPressure_bar_Inproc : FVT_lib/outp/OverrideAndLimit  SystemSampleTime=-1  VariantActivationTime=update diagram  Latency=0  AutoFrameSizeCalculation=off
      link override Signal_Limit/_maxval: Value=KOUTP_MCPressure_bar_maxval
      link override Signal_Limit/_minval: Value=KOUTP_MCPressure_bar_minval
      link override Signal_Override/_ovrdflg: Value=KOUTP_MCPressure_bar_ovrdflg
      link override Signal_Override/_ovrdval: Value=KOUTP_MCPressure_bar_ovrdval
  VAPM_ModOperation_enum_Inproc : FVT_lib/outp/OverrideAndLimit  SystemSampleTime=-1  VariantActivationTime=update diagram  Latency=0  AutoFrameSizeCalculation=off
      link override Signal_Limit/_maxval: Value=KOUTP_ModOperation_enum_maxval
      link override Signal_Limit/_minval: Value=KOUTP_ModOperation_enum_minval
      link override Signal_Override/_ovrdflg: Value=KOUTP_ModOperation_enum_ovrdflg
      link override Signal_Override/_ovrdval: Value=KOUTP_ModOperation_enum_ovrdval
  VAPM_PASAFCL_enum_Inproc : FVT_lib/outp/OverrideAndLimit  SystemSampleTime=-1  VariantActivationTime=update diagram  Latency=0  AutoFrameSizeCalculation=off
      link override Signal_Limit/_maxval: Value=KOUTP_PASAFCL_enum_maxval
      link override Signal_Limit/_minval: Value=KOUTP_PASAFCL_enum_minval
      link override Signal_Override/_ovrdflg: Value=KOUTP_PASAFCL_enum_ovrdflg
      link override Signal_Override/_ovrdval: Value=KOUTP_PASAFCL_enum_ovrdval
  VAPM_PASAFCR_enum_Inproc : FVT_lib/outp/OverrideAndLimit  SystemSampleTime=-1  VariantActivationTime=update diagram  Latency=0  AutoFrameSizeCalculation=off
      link override Signal_Limit/_maxval: Value=KOUTP_PASAFCR_enum_maxval
      link override Signal_Limit/_minval: Value=KOUTP_PASAFCR_enum_minval
      link override Signal_Override/_ovrdflg: Value=KOUTP_PASAFCR_enum_ovrdflg
      link override Signal_Override/_ovrdval: Value=KOUTP_PASAFCR_enum_ovrdval
  VAPM_PASAFML_enum_Inproc : FVT_lib/outp/OverrideAndLimit  SystemSampleTime=-1  VariantActivationTime=update diagram  Latency=0  AutoFrameSizeCalculation=off
      link override Signal_Limit/_maxval: Value=KOUTP_PASAFML_enum_maxval
      link override Signal_Limit/_minval: Value=KOUTP_PASAFML_enum_minval
      link override Signal_Override/_ovrdflg: Value=KOUTP_PASAFML_enum_ovrdflg
      link override Signal_Override/_ovrdval: Value=KOUTP_PASAFML_enum_ovrdval
  VAPM_PASAFMR_enum_Inproc : FVT_lib/outp/OverrideAndLimit  SystemSampleTime=-1  VariantActivationTime=update diagram  Latency=0  AutoFrameSizeCalculation=off
      link override Signal_Limit/_maxval: Value=KOUTP_PASAFMR_enum_maxval
      link override Signal_Limit/_minval: Value=KOUTP_PASAFMR_enum_minval
      link override Signal_Override/_ovrdflg: Value=KOUTP_PASAFMR_enum_ovrdflg
      link override Signal_Override/_ovrdval: Value=KOUTP_PASAFMR_enum_ovrdval
  VAPM_PASARCL_enum_Inproc : FVT_lib/outp/OverrideAndLimit  SystemSampleTime=-1  VariantActivationTime=update diagram  Latency=0  AutoFrameSizeCalculation=off
      link override Signal_Limit/_maxval: Value=KOUTP_PASARCL_enum_maxval
      link override Signal_Limit/_minval: Value=KOUTP_PASARCL_enum_minval
      link override Signal_Override/_ovrdflg: Value=KOUTP_PASARCL_enum_ovrdflg
      link override Signal_Override/_ovrdval: Value=KOUTP_PASARCL_enum_ovrdval
  VAPM_PASARCR_enum_Inproc : FVT_lib/outp/OverrideAndLimit  SystemSampleTime=-1  VariantActivationTime=update diagram  Latency=0  AutoFrameSizeCalculation=off
      link override Signal_Limit/_maxval: Value=KOUTP_PASARCR_enum_maxval
      link override Signal_Limit/_minval: Value=KOUTP_PASARCR_enum_minval
      link override Signal_Override/_ovrdflg: Value=KOUTP_PASARCR_enum_ovrdflg
      link override Signal_Override/_ovrdval: Value=KOUTP_PASARCR_enum_ovrdval
  VAPM_PASARML_enum_Inproc : FVT_lib/outp/OverrideAndLimit  SystemSampleTime=-1  VariantActivationTime=update diagram  Latency=0  AutoFrameSizeCalculation=off
      link override Signal_Limit/_maxval: Value=KOUTP_PASARML_enum_maxval
      link override Signal_Limit/_minval: Value=KOUTP_PASARML_enum_minval
      link override Signal_Override/_ovrdflg: Value=KOUTP_PASARML_enum_ovrdflg
      link override Signal_Override/_ovrdval: Value=KOUTP_PASARML_enum_ovrdval
  VAPM_PASARMR_enum_Inproc : FVT_lib/outp/OverrideAndLimit  SystemSampleTime=-1  VariantActivationTime=update diagram  Latency=0  AutoFrameSizeCalculation=off
      link override Signal_Limit/_maxval: Value=KOUTP_PASARMR_enum_maxval
      link override Signal_Limit/_minval: Value=KOUTP_PASARMR_enum_minval
      link override Signal_Override/_ovrdflg: Value=KOUTP_PASARMR_enum_ovrdflg
      link override Signal_Override/_ovrdval: Value=KOUTP_PASARMR_enum_ovrdval
  VAPM_PASDFCL_cm_Inproc : FVT_lib/outp/OverrideAndLimit  SystemSampleTime=-1  VariantActivationTime=update diagram  Latency=0  AutoFrameSizeCalculation=off
      link override Signal_Limit/_maxval: Value=KOUTP_PASDFCL_cm_maxval
      link override Signal_Limit/_minval: Value=KOUTP_PASDFCL_cm_minval
      link override Signal_Override/_ovrdflg: Value=KOUTP_PASDFCL_cm_ovrdflg
      link override Signal_Override/_ovrdval: Value=KOUTP_PASDFCL_cm_ovrdval
  VAPM_PASDFCR_cm_Inproc : FVT_lib/outp/OverrideAndLimit  SystemSampleTime=-1  VariantActivationTime=update diagram  Latency=0  AutoFrameSizeCalculation=off
      link override Signal_Limit/_maxval: Value=KOUTP_PASDFCR_cm_maxval
      link override Signal_Limit/_minval: Value=KOUTP_PASDFCR_cm_minval
      link override Signal_Override/_ovrdflg: Value=KOUTP_PASDFCR_cm_ovrdflg
      link override Signal_Override/_ovrdval: Value=KOUTP_PASDFCR_cm_ovrdval
  VAPM_PASDFML_cm_Inproc : FVT_lib/outp/OverrideAndLimit  SystemSampleTime=-1  VariantActivationTime=update diagram  Latency=0  AutoFrameSizeCalculation=off
      link override Signal_Limit/_maxval: Value=KOUTP_PASDFML_cm_maxval
      link override Signal_Limit/_minval: Value=KOUTP_PASDFML_cm_minval
      link override Signal_Override/_ovrdflg: Value=KOUTP_PASDFML_cm_ovrdflg
      link override Signal_Override/_ovrdval: Value=KOUTP_PASDFML_cm_ovrdval
  VAPM_PASDFMR_cm_Inproc : FVT_lib/outp/OverrideAndLimit  SystemSampleTime=-1  VariantActivationTime=update diagram  Latency=0  AutoFrameSizeCalculation=off
      link override Signal_Limit/_maxval: Value=KOUTP_PASDFMR_cm_maxval
      link override Signal_Limit/_minval: Value=KOUTP_PASDFMR_cm_minval
      link override Signal_Override/_ovrdflg: Value=KOUTP_PASDFMR_cm_ovrdflg
      link override Signal_Override/_ovrdval: Value=KOUTP_PASDFMR_cm_ovrdval
  VAPM_PASDRCL_cm_Inproc : FVT_lib/outp/OverrideAndLimit  SystemSampleTime=-1  VariantActivationTime=update diagram  Latency=0  AutoFrameSizeCalculation=off
      link override Signal_Limit/_maxval: Value=KOUTP_PASDRCL_cm_maxval
      link override Signal_Limit/_minval: Value=KOUTP_PASDRCL_cm_minval
      link override Signal_Override/_ovrdflg: Value=KOUTP_PASDRCL_cm_ovrdflg
      link override Signal_Override/_ovrdval: Value=KOUTP_PASDRCL_cm_ovrdval
  VAPM_PASDRCR_cm_Inproc : FVT_lib/outp/OverrideAndLimit  SystemSampleTime=-1  VariantActivationTime=update diagram  Latency=0  AutoFrameSizeCalculation=off
      link override Signal_Limit/_maxval: Value=KOUTP_PASDRCR_cm_maxval
      link override Signal_Limit/_minval: Value=KOUTP_PASDRCR_cm_minval
      link override Signal_Override/_ovrdflg: Value=KOUTP_PASDRCR_cm_ovrdflg
      link override Signal_Override/_ovrdval: Value=KOUTP_PASDRCR_cm_ovrdval
  VAPM_PASDRML_cm_Inproc : FVT_lib/outp/OverrideAndLimit  SystemSampleTime=-1  VariantActivationTime=update diagram  Latency=0  AutoFrameSizeCalculation=off
      link override Signal_Limit/_maxval: Value=KOUTP_PASDRML_cm_maxval
      link override Signal_Limit/_minval: Value=KOUTP_PASDRML_cm_minval
      link override Signal_Override/_ovrdflg: Value=KOUTP_PASDRML_cm_ovrdflg
      link override Signal_Override/_ovrdval: Value=KOUTP_PASDRML_cm_ovrdval
  VAPM_PASDRMR_cm_Inproc : FVT_lib/outp/OverrideAndLimit  SystemSampleTime=-1  VariantActivationTime=update diagram  Latency=0  AutoFrameSizeCalculation=off
      link override Signal_Limit/_maxval: Value=KOUTP_PASDRMR_cm_maxval
      link override Signal_Limit/_minval: Value=KOUTP_PASDRMR_cm_minval
      link override Signal_Override/_ovrdflg: Value=KOUTP_PASDRMR_cm_ovrdflg
      link override Signal_Override/_ovrdval: Value=KOUTP_PASDRMR_cm_ovrdval
  VAPM_PUIDLowPower_flg_Inproc : FVT_lib/outp/OverrideAndLimit  SystemSampleTime=-1  VariantActivationTime=update diagram  Latency=0  AutoFrameSizeCalculation=off
      link override Signal_Limit/_maxval: Value=KOUTP_PUIDLowPower_flg_maxval
      link override Signal_Limit/_minval: Value=KOUTP_PUIDLowPower_flg_minval
      link override Signal_Override/_ovrdflg: Value=KOUTP_PUIDLowPower_flg_ovrdflg
      link override Signal_Override/_ovrdval: Value=KOUTP_PUIDLowPower_flg_ovrdval
  VAPM_RAPSBCMLamp_enum_Inproc : FVT_lib/outp/OverrideAndLimit  SystemSampleTime=-1  VariantActivationTime=update diagram  Latency=0  AutoFrameSizeCalculation=off
      link override Signal_Limit/_maxval: Value=KOUTP_RAPSBCMLamp_enum_maxval
      link override Signal_Limit/_minval: Value=KOUTP_RAPSBCMLamp_enum_minval
      link override Signal_Override/_ovrdflg: Value=KOUTP_RAPSBCMLamp_enum_ovrdflg
      link override Signal_Override/_ovrdval: Value=KOUTP_RAPSBCMLamp_enum_ovrdval
  VAPM_RAPSBCMLockReq_flg_Inproc : FVT_lib/outp/OverrideAndLimit  SystemSampleTime=-1  VariantActivationTime=update diagram  Latency=0  AutoFrameSizeCalculation=off
      link override Signal_Limit/_maxval: Value=KOUTP_RAPSBCMLockReq_flg_maxval
      link override Signal_Limit/_minval: Value=KOUTP_RAPSBCMLockReq_flg_minval
      link override Signal_Override/_ovrdflg: Value=KOUTP_RAPSBCMLockReq_flg_ovrdflg
      link override Signal_Override/_ovrdval: Value=KOUTP_RAPSBCMLockReq_flg_ovrdval
  VAPM_RAPSErrLv1_flg_Inproc : FVT_lib/outp/OverrideAndLimit  SystemSampleTime=-1  VariantActivationTime=update diagram  Latency=0  AutoFrameSizeCalculation=off
      link override Signal_Limit/_maxval: Value=KOUTP_RAPSErrLv1_flg_maxval
      link override Signal_Limit/_minval: Value=KOUTP_RAPSErrLv1_flg_minval
      link override Signal_Override/_ovrdflg: Value=KOUTP_RAPSErrLv1_flg_ovrdflg
      link override Signal_Override/_ovrdval: Value=KOUTP_RAPSErrLv1_flg_ovrdval
  VAPM_RAPSErrWarnSta_enum_Inproc : FVT_lib/outp/OverrideAndLimit  SystemSampleTime=-1  VariantActivationTime=update diagram  Latency=0  AutoFrameSizeCalculation=off
      link override Signal_Limit/_maxval: Value=KOUTP_RAPSErrWarnSta_enum_maxval
      link override Signal_Limit/_minval: Value=KOUTP_RAPSErrWarnSta_enum_minval
      link override Signal_Override/_ovrdflg: Value=KOUTP_RAPSErrWarnSta_enum_ovrdflg
      link override Signal_Override/_ovrdval: Value=KOUTP_RAPSErrWarnSta_enum_ovrdval
  VAPM_RFPulseCountTimeOut_flg_Inproc : FVT_lib/outp/OverrideAndLimit  SystemSampleTime=-1  VariantActivationTime=update diagram  Latency=0  AutoFrameSizeCalculation=off
      link override Signal_Limit/_maxval: Value=KOUTP_RFPulseCountTimeOut_flg_maxval
      link override Signal_Limit/_minval: Value=KOUTP_RFPulseCountTimeOut_flg_minval
      link override Signal_Override/_ovrdflg: Value=KOUTP_RFPulseCountTimeOut_flg_ovrdflg
      link override Signal_Override/_ovrdval: Value=KOUTP_RFPulseCountTimeOut_flg_ovrdval
  VAPM_RFPulseCountVTimeOut_flg_Inproc : FVT_lib/outp/OverrideAndLimit  SystemSampleTime=-1  VariantActivationTime=update diagram  Latency=0  AutoFrameSizeCalculation=off
      link override Signal_Limit/_maxval: Value=KOUTP_RFPulseCountVTimeOut_flg_maxval
      link override Signal_Limit/_minval: Value=KOUTP_RFPulseCountVTimeOut_flg_minval
      link override Signal_Override/_ovrdflg: Value=KOUTP_RFPulseCountVTimeOut_flg_ovrdflg
      link override Signal_Override/_ovrdval: Value=KOUTP_RFPulseCountVTimeOut_flg_ovrdval
  VAPM_RFPulseCountV_flg_Inproc : FVT_lib/outp/OverrideAndLimit  SystemSampleTime=-1  VariantActivationTime=update diagram  Latency=0  AutoFrameSizeCalculation=off
      link override Signal_Limit/_maxval: Value=KOUTP_RFPulseCountV_flg_maxval
      link override Signal_Limit/_minval: Value=KOUTP_RFPulseCountV_flg_minval
      link override Signal_Override/_ovrdflg: Value=KOUTP_RFPulseCountV_flg_ovrdflg
      link override Signal_Override/_ovrdval: Value=KOUTP_RFPulseCountV_flg_ovrdval
  VAPM_RFPulseCount_enum_Inproc : FVT_lib/outp/OverrideAndLimit  SystemSampleTime=-1  VariantActivationTime=update diagram  Latency=0  AutoFrameSizeCalculation=off
      link override Signal_Limit/_maxval: Value=KOUTP_RFPulseCount_enum_maxval
      link override Signal_Limit/_minval: Value=KOUTP_RFPulseCount_enum_minval
      link override Signal_Override/_ovrdflg: Value=KOUTP_RFPulseCount_enum_ovrdflg
      link override Signal_Override/_ovrdval: Value=KOUTP_RFPulseCount_enum_ovrdval
  VAPM_RFRawWhlSpeedTimeOut_flg_Inproc : FVT_lib/outp/OverrideAndLimit  SystemSampleTime=-1  VariantActivationTime=update diagram  Latency=0  AutoFrameSizeCalculation=off
      link override Signal_Limit/_maxval: Value=KOUTP_RFRawWhlSpeedTimeOut_flg_maxval
      link override Signal_Limit/_minval: Value=KOUTP_RFRawWhlSpeedTimeOut_flg_minval
      link override Signal_Override/_ovrdflg: Value=KOUTP_RFRawWhlSpeedTimeOut_flg_ovrdflg
      link override Signal_Override/_ovrdval: Value=KOUTP_RFRawWhlSpeedTimeOut_flg_ovrdval
  VAPM_RFRawWhlSpeedVTimeOut_flg_Inproc : FVT_lib/outp/OverrideAndLimit  SystemSampleTime=-1  VariantActivationTime=update diagram  Latency=0  AutoFrameSizeCalculation=off
      link override Signal_Limit/_maxval: Value=KOUTP_RFRawWhlSpeedVTimeOut_flg_maxval
      link override Signal_Limit/_minval: Value=KOUTP_RFRawWhlSpeedVTimeOut_flg_minval
      link override Signal_Override/_ovrdflg: Value=KOUTP_RFRawWhlSpeedVTimeOut_flg_ovrdflg
      link override Signal_Override/_ovrdval: Value=KOUTP_RFRawWhlSpeedVTimeOut_flg_ovrdval
  VAPM_RFRawWhlSpeedV_flg_Inproc : FVT_lib/outp/OverrideAndLimit  SystemSampleTime=-1  VariantActivationTime=update diagram  Latency=0  AutoFrameSizeCalculation=off
      link override Signal_Limit/_maxval: Value=KOUTP_RFRawWhlSpeedV_flg_maxval
      link override Signal_Limit/_minval: Value=KOUTP_RFRawWhlSpeedV_flg_minval
      link override Signal_Override/_ovrdflg: Value=KOUTP_RFRawWhlSpeedV_flg_ovrdflg
      link override Signal_Override/_ovrdval: Value=KOUTP_RFRawWhlSpeedV_flg_ovrdval
  VAPM_RFRawWhlSpeed_kph_Inproc : FVT_lib/outp/OverrideAndLimit  SystemSampleTime=-1  VariantActivationTime=update diagram  Latency=0  AutoFrameSizeCalculation=off
      link override Signal_Limit/_maxval: Value=KOUTP_RFRawWhlSpeed_kph_maxval
      link override Signal_Limit/_minval: Value=KOUTP_RFRawWhlSpeed_kph_minval
      link override Signal_Override/_ovrdflg: Value=KOUTP_RFRawWhlSpeed_kph_ovrdflg
      link override Signal_Override/_ovrdval: Value=KOUTP_RFRawWhlSpeed_kph_ovrdval
  VAPM_RFWhlRotDirTimeOut_flg_Inproc : FVT_lib/outp/OverrideAndLimit  SystemSampleTime=-1  VariantActivationTime=update diagram  Latency=0  AutoFrameSizeCalculation=off
      link override Signal_Limit/_maxval: Value=KOUTP_RFWhlRotDirTimeOut_flg_maxval
      link override Signal_Limit/_minval: Value=KOUTP_RFWhlRotDirTimeOut_flg_minval
      link override Signal_Override/_ovrdflg: Value=KOUTP_RFWhlRotDirTimeOut_flg_ovrdflg
      link override Signal_Override/_ovrdval: Value=KOUTP_RFWhlRotDirTimeOut_flg_ovrdval
  VAPM_RFWhlRotDir_enum_Inproc : FVT_lib/outp/OverrideAndLimit  SystemSampleTime=-1  VariantActivationTime=update diagram  Latency=0  AutoFrameSizeCalculation=off
      link override Signal_Limit/_maxval: Value=KOUTP_RFWhlRotDir_enum_maxval
      link override Signal_Limit/_minval: Value=KOUTP_RFWhlRotDir_enum_minval
      link override Signal_Override/_ovrdflg: Value=KOUTP_RFWhlRotDir_enum_ovrdflg
      link override Signal_Override/_ovrdval: Value=KOUTP_RFWhlRotDir_enum_ovrdval
  VAPM_RRPulseCountTimeOut_flg_Inproc : FVT_lib/outp/OverrideAndLimit  SystemSampleTime=-1  VariantActivationTime=update diagram  Latency=0  AutoFrameSizeCalculation=off
      link override Signal_Limit/_maxval: Value=KOUTP_RRPulseCountTimeOut_flg_maxval
      link override Signal_Limit/_minval: Value=KOUTP_RRPulseCountTimeOut_flg_minval
      link override Signal_Override/_ovrdflg: Value=KOUTP_RRPulseCountTimeOut_flg_ovrdflg
      link override Signal_Override/_ovrdval: Value=KOUTP_RRPulseCountTimeOut_flg_ovrdval
  VAPM_RRPulseCountVTimeOut_flg_Inproc : FVT_lib/outp/OverrideAndLimit  SystemSampleTime=-1  VariantActivationTime=update diagram  Latency=0  AutoFrameSizeCalculation=off
      link override Signal_Limit/_maxval: Value=KOUTP_RRPulseCountVTimeOut_flg_maxval
      link override Signal_Limit/_minval: Value=KOUTP_RRPulseCountVTimeOut_flg_minval
      link override Signal_Override/_ovrdflg: Value=KOUTP_RRPulseCountVTimeOut_flg_ovrdflg
      link override Signal_Override/_ovrdval: Value=KOUTP_RRPulseCountVTimeOut_flg_ovrdval
  VAPM_RRPulseCountV_flg_Inproc : FVT_lib/outp/OverrideAndLimit  SystemSampleTime=-1  VariantActivationTime=update diagram  Latency=0  AutoFrameSizeCalculation=off
      link override Signal_Limit/_maxval: Value=KOUTP_RRPulseCountV_flg_maxval
      link override Signal_Limit/_minval: Value=KOUTP_RRPulseCountV_flg_minval
      link override Signal_Override/_ovrdflg: Value=KOUTP_RRPulseCountV_flg_ovrdflg
      link override Signal_Override/_ovrdval: Value=KOUTP_RRPulseCountV_flg_ovrdval
  VAPM_RRPulseCount_enum_Inproc : FVT_lib/outp/OverrideAndLimit  SystemSampleTime=-1  VariantActivationTime=update diagram  Latency=0  AutoFrameSizeCalculation=off
      link override Signal_Limit/_maxval: Value=KOUTP_RRPulseCount_enum_maxval
      link override Signal_Limit/_minval: Value=KOUTP_RRPulseCount_enum_minval
      link override Signal_Override/_ovrdflg: Value=KOUTP_RRPulseCount_enum_ovrdflg
      link override Signal_Override/_ovrdval: Value=KOUTP_RRPulseCount_enum_ovrdval
  VAPM_RRRawWhlSpeedTimeOut_flg_Inproc : FVT_lib/outp/OverrideAndLimit  SystemSampleTime=-1  VariantActivationTime=update diagram  Latency=0  AutoFrameSizeCalculation=off
      link override Signal_Limit/_maxval: Value=KOUTP_RRRawWhlSpeedTimeOut_flg_maxval
      link override Signal_Limit/_minval: Value=KOUTP_RRRawWhlSpeedTimeOut_flg_minval
      link override Signal_Override/_ovrdflg: Value=KOUTP_RRRawWhlSpeedTimeOut_flg_ovrdflg
      link override Signal_Override/_ovrdval: Value=KOUTP_RRRawWhlSpeedTimeOut_flg_ovrdval
  VAPM_RRRawWhlSpeedVTimeOut_flg_Inproc : FVT_lib/outp/OverrideAndLimit  SystemSampleTime=-1  VariantActivationTime=update diagram  Latency=0  AutoFrameSizeCalculation=off
      link override Signal_Limit/_maxval: Value=KOUTP_RRRawWhlSpeedVTimeOut_flg_maxval
      link override Signal_Limit/_minval: Value=KOUTP_RRRawWhlSpeedVTimeOut_flg_minval
      link override Signal_Override/_ovrdflg: Value=KOUTP_RRRawWhlSpeedVTimeOut_flg_ovrdflg
      link override Signal_Override/_ovrdval: Value=KOUTP_RRRawWhlSpeedVTimeOut_flg_ovrdval
  VAPM_RRRawWhlSpeedV_flg_Inproc : FVT_lib/outp/OverrideAndLimit  SystemSampleTime=-1  VariantActivationTime=update diagram  Latency=0  AutoFrameSizeCalculation=off
      link override Signal_Limit/_maxval: Value=KOUTP_RRRawWhlSpeedV_flg_maxval
      link override Signal_Limit/_minval: Value=KOUTP_RRRawWhlSpeedV_flg_minval
      link override Signal_Override/_ovrdflg: Value=KOUTP_RRRawWhlSpeedV_flg_ovrdflg
      link override Signal_Override/_ovrdval: Value=KOUTP_RRRawWhlSpeedV_flg_ovrdval
  VAPM_RRRawWhlSpeed_kph_Inproc : FVT_lib/outp/OverrideAndLimit  SystemSampleTime=-1  VariantActivationTime=update diagram  Latency=0  AutoFrameSizeCalculation=off
      link override Signal_Limit/_maxval: Value=KOUTP_RRRawWhlSpeed_kph_maxval
      link override Signal_Limit/_minval: Value=KOUTP_RRRawWhlSpeed_kph_minval
      link override Signal_Override/_ovrdflg: Value=KOUTP_RRRawWhlSpeed_kph_ovrdflg
      link override Signal_Override/_ovrdval: Value=KOUTP_RRRawWhlSpeed_kph_ovrdval
  VAPM_RRWhlRotDirTimeOut_flg_Inproc : FVT_lib/outp/OverrideAndLimit  SystemSampleTime=-1  VariantActivationTime=update diagram  Latency=0  AutoFrameSizeCalculation=off
      link override Signal_Limit/_maxval: Value=KOUTP_RRWhlRotDirTimeOut_flg_maxval
      link override Signal_Limit/_minval: Value=KOUTP_RRWhlRotDirTimeOut_flg_minval
      link override Signal_Override/_ovrdflg: Value=KOUTP_RRWhlRotDirTimeOut_flg_ovrdflg
      link override Signal_Override/_ovrdval: Value=KOUTP_RRWhlRotDirTimeOut_flg_ovrdval
  VAPM_RRWhlRotDir_enum_Inproc : FVT_lib/outp/OverrideAndLimit  SystemSampleTime=-1  VariantActivationTime=update diagram  Latency=0  AutoFrameSizeCalculation=off
      link override Signal_Limit/_maxval: Value=KOUTP_RRWhlRotDir_enum_maxval
      link override Signal_Limit/_minval: Value=KOUTP_RRWhlRotDir_enum_minval
      link override Signal_Override/_ovrdflg: Value=KOUTP_RRWhlRotDir_enum_ovrdflg
      link override Signal_Override/_ovrdval: Value=KOUTP_RRWhlRotDir_enum_ovrdval
  VAPM_SASAngleTimeOut_flg_Inproc : FVT_lib/outp/OverrideAndLimit  SystemSampleTime=-1  VariantActivationTime=update diagram  Latency=0  AutoFrameSizeCalculation=off
      link override Signal_Limit/_maxval: Value=KOUTP_SASAngleTimeOut_flg_maxval
      link override Signal_Limit/_minval: Value=KOUTP_SASAngleTimeOut_flg_minval
      link override Signal_Override/_ovrdflg: Value=KOUTP_SASAngleTimeOut_flg_ovrdflg
      link override Signal_Override/_ovrdval: Value=KOUTP_SASAngleTimeOut_flg_ovrdval
  VAPM_SASAngle_Deg_Inproc : FVT_lib/outp/OverrideAndLimit  SystemSampleTime=-1  VariantActivationTime=update diagram  Latency=0  AutoFrameSizeCalculation=off
      link override Signal_Limit/_maxval: Value=KOUTP_SASAngle_Deg_maxval
      link override Signal_Limit/_minval: Value=KOUTP_SASAngle_Deg_minval
      link override Signal_Override/_ovrdflg: Value=KOUTP_SASAngle_Deg_ovrdflg
      link override Signal_Override/_ovrdval: Value=KOUTP_SASAngle_Deg_ovrdval
  VAPM_SASCALTimeOut_flg_Inproc : FVT_lib/outp/OverrideAndLimit  SystemSampleTime=-1  VariantActivationTime=update diagram  Latency=0  AutoFrameSizeCalculation=off
      link override Signal_Limit/_maxval: Value=KOUTP_SASCALTimeOut_flg_maxval
      link override Signal_Limit/_minval: Value=KOUTP_SASCALTimeOut_flg_minval
      link override Signal_Override/_ovrdflg: Value=KOUTP_SASCALTimeOut_flg_ovrdflg
      link override Signal_Override/_ovrdval: Value=KOUTP_SASCALTimeOut_flg_ovrdval
  VAPM_SASCAL_flg_Inproc : FVT_lib/outp/OverrideAndLimit  SystemSampleTime=-1  VariantActivationTime=update diagram  Latency=0  AutoFrameSizeCalculation=off
      link override Signal_Limit/_maxval: Value=KOUTP_SASCAL_flg_maxval
      link override Signal_Limit/_minval: Value=KOUTP_SASCAL_flg_minval
      link override Signal_Override/_ovrdflg: Value=KOUTP_SASCAL_flg_ovrdflg
      link override Signal_Override/_ovrdval: Value=KOUTP_SASCAL_flg_ovrdval
  VAPM_SASSpeedTimeOut_flg_Inproc : FVT_lib/outp/OverrideAndLimit  SystemSampleTime=-1  VariantActivationTime=update diagram  Latency=0  AutoFrameSizeCalculation=off
      link override Signal_Limit/_maxval: Value=KOUTP_SASSpeedTimeOut_flg_maxval
      link override Signal_Limit/_minval: Value=KOUTP_SASSpeedTimeOut_flg_minval
      link override Signal_Override/_ovrdflg: Value=KOUTP_SASSpeedTimeOut_flg_ovrdflg
      link override Signal_Override/_ovrdval: Value=KOUTP_SASSpeedTimeOut_flg_ovrdval
  VAPM_SASSpeedValidTimeOut_flg_Inproc : FVT_lib/outp/OverrideAndLimit  SystemSampleTime=-1  VariantActivationTime=update diagram  Latency=0  AutoFrameSizeCalculation=off
      link override Signal_Limit/_maxval: Value=KOUTP_SASSpeedValidTimeOut_flg_maxval
      link override Signal_Limit/_minval: Value=KOUTP_SASSpeedValidTimeOut_flg_minval
      link override Signal_Override/_ovrdflg: Value=KOUTP_SASSpeedValidTimeOut_flg_ovrdflg
      link override Signal_Override/_ovrdval: Value=KOUTP_SASSpeedValidTimeOut_flg_ovrdval
  VAPM_SASSpeedValid_flg_Inproc : FVT_lib/outp/OverrideAndLimit  SystemSampleTime=-1  VariantActivationTime=update diagram  Latency=0  AutoFrameSizeCalculation=off
      link override Signal_Limit/_maxval: Value=KOUTP_SASSpeedValid_flg_maxval
      link override Signal_Limit/_minval: Value=KOUTP_SASSpeedValid_flg_minval
      link override Signal_Override/_ovrdflg: Value=KOUTP_SASSpeedValid_flg_ovrdflg
      link override Signal_Override/_ovrdval: Value=KOUTP_SASSpeedValid_flg_ovrdval
  VAPM_SASSpeed_degps_Inproc : FVT_lib/outp/OverrideAndLimit  SystemSampleTime=-1  VariantActivationTime=update diagram  Latency=0  AutoFrameSizeCalculation=off
      link override Signal_Limit/_maxval: Value=KOUTP_SASSpeed_degps_maxval
      link override Signal_Limit/_minval: Value=KOUTP_SASSpeed_degps_minval
      link override Signal_Override/_ovrdflg: Value=KOUTP_SASSpeed_degps_ovrdflg
      link override Signal_Override/_ovrdval: Value=KOUTP_SASSpeed_degps_ovrdval
  VAPM_SASVTimeOut_flg_Inproc : FVT_lib/outp/OverrideAndLimit  SystemSampleTime=-1  VariantActivationTime=update diagram  Latency=0  AutoFrameSizeCalculation=off
      link override Signal_Limit/_maxval: Value=KOUTP_SASVTimeOut_flg_maxval
      link override Signal_Limit/_minval: Value=KOUTP_SASVTimeOut_flg_minval
      link override Signal_Override/_ovrdflg: Value=KOUTP_SASVTimeOut_flg_ovrdflg
      link override Signal_Override/_ovrdval: Value=KOUTP_SASVTimeOut_flg_ovrdval
  VAPM_SASV_flg_Inproc : FVT_lib/outp/OverrideAndLimit  SystemSampleTime=-1  VariantActivationTime=update diagram  Latency=0  AutoFrameSizeCalculation=off
      link override Signal_Limit/_maxval: Value=KOUTP_SASV_flg_maxval
      link override Signal_Limit/_minval: Value=KOUTP_SASV_flg_minval
      link override Signal_Override/_ovrdflg: Value=KOUTP_SASV_flg_ovrdflg
      link override Signal_Override/_ovrdval: Value=KOUTP_SASV_flg_ovrdval
  VAPM_SNSRLayout_enum_Inproc : FVT_lib/outp/OverrideAndLimit  SystemSampleTime=-1  VariantActivationTime=update diagram  Latency=0  AutoFrameSizeCalculation=off
      link override Signal_Limit/_maxval: Value=KOUTP_SNSRLayout_enum_maxval
      link override Signal_Limit/_minval: Value=KOUTP_SNSRLayout_enum_minval
      link override Signal_Override/_ovrdflg: Value=KOUTP_SNSRLayout_enum_ovrdflg
      link override Signal_Override/_ovrdval: Value=KOUTP_SNSRLayout_enum_ovrdval
  VAPM_ShifterHandleCmdTimeOut_flg_Inproc : FVT_lib/outp/OverrideAndLimit  SystemSampleTime=-1  VariantActivationTime=update diagram  Latency=0  AutoFrameSizeCalculation=off
      link override Signal_Limit/_maxval: Value=KOUTP_ShifterHandleCmdTimeOut_flg_maxval
      link override Signal_Limit/_minval: Value=KOUTP_ShifterHandleCmdTimeOut_flg_minval
      link override Signal_Override/_ovrdflg: Value=KOUTP_ShifterHandleCmdTimeOut_flg_ovrdflg
      link override Signal_Override/_ovrdval: Value=KOUTP_ShifterHandleCmdTimeOut_flg_ovrdval
  VAPM_ShifterHandleCmd_enum_Inproc : FVT_lib/outp/OverrideAndLimit  SystemSampleTime=-1  VariantActivationTime=update diagram  Latency=0  AutoFrameSizeCalculation=off
      link override Signal_Limit/_maxval: Value=KOUTP_ShifterHandleCmd_enum_maxval
      link override Signal_Limit/_minval: Value=KOUTP_ShifterHandleCmd_enum_minval
      link override Signal_Override/_ovrdflg: Value=KOUTP_ShifterHandleCmd_enum_ovrdflg
      link override Signal_Override/_ovrdval: Value=KOUTP_ShifterHandleCmd_enum_ovrdval
  VAPM_StaFSya_flg_Inproc : FVT_lib/outp/OverrideAndLimit  SystemSampleTime=-1  VariantActivationTime=update diagram  Latency=0  AutoFrameSizeCalculation=off
      link override Signal_Limit/_maxval: Value=KOUTP_StaFSya_flg_maxval
      link override Signal_Limit/_minval: Value=KOUTP_StaFSya_flg_minval
      link override Signal_Override/_ovrdflg: Value=KOUTP_StaFSya_flg_ovrdflg
      link override Signal_Override/_ovrdval: Value=KOUTP_StaFSya_flg_ovrdval
  VAPM_TCSActiveTimeOut_flg_Inproc : FVT_lib/outp/OverrideAndLimit  SystemSampleTime=-1  VariantActivationTime=update diagram  Latency=0  AutoFrameSizeCalculation=off
      link override Signal_Limit/_maxval: Value=KOUTP_TCSActiveTimeOut_flg_maxval
      link override Signal_Limit/_minval: Value=KOUTP_TCSActiveTimeOut_flg_minval
      link override Signal_Override/_ovrdflg: Value=KOUTP_TCSActiveTimeOut_flg_ovrdflg
      link override Signal_Override/_ovrdval: Value=KOUTP_TCSActiveTimeOut_flg_ovrdval
  VAPM_TCSActive_flg_Inproc : FVT_lib/outp/OverrideAndLimit  SystemSampleTime=-1  VariantActivationTime=update diagram  Latency=0  AutoFrameSizeCalculation=off
      link override Signal_Limit/_maxval: Value=KOUTP_TCSActive_flg_maxval
      link override Signal_Limit/_minval: Value=KOUTP_TCSActive_flg_minval
      link override Signal_Override/_ovrdflg: Value=KOUTP_TCSActive_flg_ovrdflg
      link override Signal_Override/_ovrdval: Value=KOUTP_TCSActive_flg_ovrdval
  VAPM_USSStaFCL_flg_Inproc : FVT_lib/outp/OverrideAndLimit  SystemSampleTime=-1  VariantActivationTime=update diagram  Latency=0  AutoFrameSizeCalculation=off
      link override Signal_Limit/_maxval: Value=KOUTP_USSStaFCL_flg_maxval
      link override Signal_Limit/_minval: Value=KOUTP_USSStaFCL_flg_minval
      link override Signal_Override/_ovrdflg: Value=KOUTP_USSStaFCL_flg_ovrdflg
      link override Signal_Override/_ovrdval: Value=KOUTP_USSStaFCL_flg_ovrdval
  VAPM_USSStaFCR_flg_Inproc : FVT_lib/outp/OverrideAndLimit  SystemSampleTime=-1  VariantActivationTime=update diagram  Latency=0  AutoFrameSizeCalculation=off
      link override Signal_Limit/_maxval: Value=KOUTP_USSStaFCR_flg_maxval
      link override Signal_Limit/_minval: Value=KOUTP_USSStaFCR_flg_minval
      link override Signal_Override/_ovrdflg: Value=KOUTP_USSStaFCR_flg_ovrdflg
      link override Signal_Override/_ovrdval: Value=KOUTP_USSStaFCR_flg_ovrdval
  VAPM_USSStaFLL_flg_Inproc : FVT_lib/outp/OverrideAndLimit  SystemSampleTime=-1  VariantActivationTime=update diagram  Latency=0  AutoFrameSizeCalculation=off
      link override Signal_Limit/_maxval: Value=KOUTP_USSStaFLL_flg_maxval
      link override Signal_Limit/_minval: Value=KOUTP_USSStaFLL_flg_minval
      link override Signal_Override/_ovrdflg: Value=KOUTP_USSStaFLL_flg_ovrdflg
      link override Signal_Override/_ovrdval: Value=KOUTP_USSStaFLL_flg_ovrdval
  VAPM_USSStaFLR_flg_Inproc : FVT_lib/outp/OverrideAndLimit  SystemSampleTime=-1  VariantActivationTime=update diagram  Latency=0  AutoFrameSizeCalculation=off
      link override Signal_Limit/_maxval: Value=KOUTP_USSStaFLR_flg_maxval
      link override Signal_Limit/_minval: Value=KOUTP_USSStaFLR_flg_minval
      link override Signal_Override/_ovrdflg: Value=KOUTP_USSStaFLR_flg_ovrdflg
      link override Signal_Override/_ovrdval: Value=KOUTP_USSStaFLR_flg_ovrdval
  VAPM_USSStaFML_flg_Inproc : FVT_lib/outp/OverrideAndLimit  SystemSampleTime=-1  VariantActivationTime=update diagram  Latency=0  AutoFrameSizeCalculation=off
      link override Signal_Limit/_maxval: Value=KOUTP_USSStaFML_flg_maxval
      link override Signal_Limit/_minval: Value=KOUTP_USSStaFML_flg_minval
      link override Signal_Override/_ovrdflg: Value=KOUTP_USSStaFML_flg_ovrdflg
      link override Signal_Override/_ovrdval: Value=KOUTP_USSStaFML_flg_ovrdval
  VAPM_USSStaFMR_flg_Inproc : FVT_lib/outp/OverrideAndLimit  SystemSampleTime=-1  VariantActivationTime=update diagram  Latency=0  AutoFrameSizeCalculation=off
      link override Signal_Limit/_maxval: Value=KOUTP_USSStaFMR_flg_maxval
      link override Signal_Limit/_minval: Value=KOUTP_USSStaFMR_flg_minval
      link override Signal_Override/_ovrdflg: Value=KOUTP_USSStaFMR_flg_ovrdflg
      link override Signal_Override/_ovrdval: Value=KOUTP_USSStaFMR_flg_ovrdval
  VAPM_USSStaRCL_flg_Inproc : FVT_lib/outp/OverrideAndLimit  SystemSampleTime=-1  VariantActivationTime=update diagram  Latency=0  AutoFrameSizeCalculation=off
      link override Signal_Limit/_maxval: Value=KOUTP_USSStaRCL_flg_maxval
      link override Signal_Limit/_minval: Value=KOUTP_USSStaRCL_flg_minval
      link override Signal_Override/_ovrdflg: Value=KOUTP_USSStaRCL_flg_ovrdflg
      link override Signal_Override/_ovrdval: Value=KOUTP_USSStaRCL_flg_ovrdval
  VAPM_USSStaRCR_flg_Inproc : FVT_lib/outp/OverrideAndLimit  SystemSampleTime=-1  VariantActivationTime=update diagram  Latency=0  AutoFrameSizeCalculation=off
      link override Signal_Limit/_maxval: Value=KOUTP_USSStaRCR_flg_maxval
      link override Signal_Limit/_minval: Value=KOUTP_USSStaRCR_flg_minval
      link override Signal_Override/_ovrdflg: Value=KOUTP_USSStaRCR_flg_ovrdflg
      link override Signal_Override/_ovrdval: Value=KOUTP_USSStaRCR_flg_ovrdval
  VAPM_USSStaRLL_flg_Inproc : FVT_lib/outp/OverrideAndLimit  SystemSampleTime=-1  VariantActivationTime=update diagram  Latency=0  AutoFrameSizeCalculation=off
      link override Signal_Limit/_maxval: Value=KOUTP_USSStaRLL_flg_maxval
      link override Signal_Limit/_minval: Value=KOUTP_USSStaRLL_flg_minval
      link override Signal_Override/_ovrdflg: Value=KOUTP_USSStaRLL_flg_ovrdflg
      link override Signal_Override/_ovrdval: Value=KOUTP_USSStaRLL_flg_ovrdval
  VAPM_USSStaRLR_flg_Inproc : FVT_lib/outp/OverrideAndLimit  SystemSampleTime=-1  VariantActivationTime=update diagram  Latency=0  AutoFrameSizeCalculation=off
      link override Signal_Limit/_maxval: Value=KOUTP_USSStaRLR_flg_maxval
      link override Signal_Limit/_minval: Value=KOUTP_USSStaRLR_flg_minval
      link override Signal_Override/_ovrdflg: Value=KOUTP_USSStaRLR_flg_ovrdflg
      link override Signal_Override/_ovrdval: Value=KOUTP_USSStaRLR_flg_ovrdval
  VAPM_USSStaRML_flg_Inproc : FVT_lib/outp/OverrideAndLimit  SystemSampleTime=-1  VariantActivationTime=update diagram  Latency=0  AutoFrameSizeCalculation=off
      link override Signal_Limit/_maxval: Value=KOUTP_USSStaRML_flg_maxval
      link override Signal_Limit/_minval: Value=KOUTP_USSStaRML_flg_minval
      link override Signal_Override/_ovrdflg: Value=KOUTP_USSStaRML_flg_ovrdflg
      link override Signal_Override/_ovrdval: Value=KOUTP_USSStaRML_flg_ovrdval
  VAPM_USSStaRMR_flg_Inproc : FVT_lib/outp/OverrideAndLimit  SystemSampleTime=-1  VariantActivationTime=update diagram  Latency=0  AutoFrameSizeCalculation=off
      link override Signal_Limit/_maxval: Value=KOUTP_USSStaRMR_flg_maxval
      link override Signal_Limit/_minval: Value=KOUTP_USSStaRMR_flg_minval
      link override Signal_Override/_ovrdflg: Value=KOUTP_USSStaRMR_flg_ovrdflg
      link override Signal_Override/_ovrdval: Value=KOUTP_USSStaRMR_flg_ovrdval
  VAPM_VehSpeedTimeOut_flg_Inproc : FVT_lib/outp/OverrideAndLimit  SystemSampleTime=-1  VariantActivationTime=update diagram  Latency=0  AutoFrameSizeCalculation=off
      link override Signal_Limit/_maxval: Value=KOUTP_VehSpeedTimeOut_flg_maxval
      link override Signal_Limit/_minval: Value=KOUTP_VehSpeedTimeOut_flg_minval
      link override Signal_Override/_ovrdflg: Value=KOUTP_VehSpeedTimeOut_flg_ovrdflg
